simulink model "ElevatorPlant_Storage_A"  (R2015b)
(part 5 of 8)

            (junction 89650) -> (junction 89649)
            (junction 89651) -> (junction 89650)
          state Max_Min_assignment
            state Min_but
              en:
              BUTTON=MIN_BUT;
            state Max_but
              en:
              BUTTON=MAX_BUT;
            state First_but
              en:
              BUTTON=BUT_1;
            state Max_but1
              en:
              MAX_BUT=2;
            state Max_but2
              en:
              MAX_BUT=1;
            state Max_but3
              en:
              MAX_BUT=0;
            state Min_but1
              en:
              MIN_BUT=1;
            state Min_but2
              en:
              MIN_BUT=2;
            state Min_but3
              en:
              MIN_BUT=3;
            state MAX
              en:
              MAX_BUT=BUT_TEMP;
            state MIN
              en:
              MIN_BUT=BUT_TEMP;
            state Updating_button_0
              en:
              BUTTON=MAX_BUT;
            state Updating_button_1
              en:
              BUTTON=MIN_BUT;
            (junction 89689) -> OpCl_doors.OpCl_2.Opening2.Button_detection.Max_Min_assignment.Min_but [order 1] : [(MAX_BUT-FLOOR)>(FLOOR-MIN_BUT)]
            OpCl_doors.OpCl_2.Opening2.Button_detection.Max_Min_assignment.Min_but -> (junction 89690)
            (junction 89691) -> (junction 89689) [order 1] : [not(FLAG_STOP) && MOTION==2 && FLAG==3]
            (default) -> (junction 89691)
            (junction 89689) -> (junction 89692) [order 2]
            (junction 89690) -> (junction 89693)
            (junction 89691) -> (junction 89694) [order 2]
            (junction 89692) -> OpCl_doors.OpCl_2.Opening2.Button_detection.Max_Min_assignment.Max_but [order 1] : [(MAX_BUT-FLOOR)<(FLOOR-MIN_BUT)]
            OpCl_doors.OpCl_2.Opening2.Button_detection.Max_Min_assignment.Max_but -> (junction 89693)
            (junction 89692) -> OpCl_doors.OpCl_2.Opening2.Button_detection.Max_Min_assignment.First_but [order 2]
            (junction 89693) -> (junction 89696)
            OpCl_doors.OpCl_2.Opening2.Button_detection.Max_Min_assignment.First_but -> (junction 89695)
            (junction 89695) -> (junction 89694)
            (junction 89696) -> (junction 89695)
            (junction 89694) -> (junction 89697)
            (junction 89698) -> (junction 89699) [order 1] : [MOTION==0]
                | {MOTION=1;
                | UPDATE=true;}
            (junction 89699) -> OpCl_doors.OpCl_2.Opening2.Button_detection.Max_Min_assignment.Max_but1 [order 1] : [BUTTON_UP(2)]
            OpCl_doors.OpCl_2.Opening2.Button_detection.Max_Min_assignment.Max_but1 -> (junction 89700)
            (junction 89697) -> (junction 89698) [order 1] : [BUTTON==FLOOR && EXTEND]
                | {EXTEND=false;}
            (junction 89697) -> (junction 89711) [order 2]
            (junction 89698) -> (junction 89703) [order 2]
            (junction 89699) -> (junction 89701) [order 2]
            (junction 89700) -> (junction 89702)
            (junction 89701) -> OpCl_doors.OpCl_2.Opening2.Button_detection.Max_Min_assignment.Max_but2 [order 1] : [BUTTON_UP(1)]
            OpCl_doors.OpCl_2.Opening2.Button_detection.Max_Min_assignment.Max_but2 -> (junction 89702)
            (junction 89701) -> OpCl_doors.OpCl_2.Opening2.Button_detection.Max_Min_assignment.Max_but3 [order 2]
            (junction 89702) -> (junction 89705)
            OpCl_doors.OpCl_2.Opening2.Button_detection.Max_Min_assignment.Max_but3 -> (junction 89704)
            (junction 89704) -> (junction 89703)
            (junction 89705) -> (junction 89704)
            (junction 89703) -> (junction 89706)
            (junction 89706) -> (junction 89707) [order 1] : [MOTION==1]
                | {MOTION=0;
                | UPDATE=true;}
            (junction 89707) -> OpCl_doors.OpCl_2.Opening2.Button_detection.Max_Min_assignment.Min_but1 [order 1] : [BUTTON_DOWN(1)]
            OpCl_doors.OpCl_2.Opening2.Button_detection.Max_Min_assignment.Min_but1 -> (junction 89708)
            (junction 89706) -> (junction 89712) [order 2]
            (junction 89707) -> (junction 89709) [order 2]
            (junction 89708) -> (junction 89710)
            (junction 89709) -> OpCl_doors.OpCl_2.Opening2.Button_detection.Max_Min_assignment.Min_but2 [order 1] : [BUTTON_DOWN(2)]
            OpCl_doors.OpCl_2.Opening2.Button_detection.Max_Min_assignment.Min_but2 -> (junction 89710)
            (junction 89709) -> OpCl_doors.OpCl_2.Opening2.Button_detection.Max_Min_assignment.Min_but3 [order 2]
            (junction 89710) -> (junction 89714)
            OpCl_doors.OpCl_2.Opening2.Button_detection.Max_Min_assignment.Min_but3 -> (junction 89713)
            (junction 89712) -> (junction 89711)
            (junction 89713) -> (junction 89712)
            (junction 89714) -> (junction 89713)
            (junction 89711) -> (junction 89716)
            OpCl_doors.OpCl_2.Opening2.Button_detection.Max_Min_assignment.MAX -> (junction 89715)
            (junction 89716) -> (junction 89717) [order 1] : [PUSHED]
            (junction 89717) -> (junction 89718) [order 1] : [not(BUT_TEMP==FLOOR) || not(MOTION==2)]
            (junction 89718) -> OpCl_doors.OpCl_2.Opening2.Button_detection.Max_Min_assignment.MAX [order 1] : [MAX_BUT<BUT_TEMP && not(UPDATE)]
            (junction 89715) -> (junction 89720)
            (junction 89716) -> (junction 89730) [order 2]
            (junction 89717) -> (junction 89723) [order 2]
            (junction 89718) -> (junction 89719) [order 2]
            (junction 89720) -> (junction 89719)
            (junction 89719) -> (junction 89721)
            (junction 89721) -> OpCl_doors.OpCl_2.Opening2.Button_detection.Max_Min_assignment.MIN [order 1] : [MIN_BUT>BUT_TEMP && not(UPDATE)]
            OpCl_doors.OpCl_2.Opening2.Button_detection.Max_Min_assignment.MIN -> (junction 89722)
            (junction 89721) -> (junction 89724) [order 2]
            (junction 89722) -> (junction 89725)
            (junction 89724) -> (junction 89723)
            (junction 89725) -> (junction 89724)
            (junction 89723) -> (junction 89726)
            (junction 89726) -> OpCl_doors.OpCl_2.Opening2.Button_detection.Max_Min_assignment.Updating_button_0 [order 1] : [MOTION==0]
            OpCl_doors.OpCl_2.Opening2.Button_detection.Max_Min_assignment.Updating_button_0 -> (junction 89727)
            (junction 89726) -> (junction 89728) [order 2]
            (junction 89727) -> (junction 89729)
            (junction 89728) -> OpCl_doors.OpCl_2.Opening2.Button_detection.Max_Min_assignment.Updating_button_1 [order 1] : [MOTION==1]
            OpCl_doors.OpCl_2.Opening2.Button_detection.Max_Min_assignment.Updating_button_1 -> (junction 89729)
            (junction 89728) -> (junction 89731) [order 2]
            (junction 89729) -> (junction 89732)
            (junction 89731) -> (junction 89730)
            (junction 89732) -> (junction 89731)
          state GoTo_PositionControl
            en:
            BUTTON=BUT_TEMP;
            FLAG=2;
          state Emergency
            en:
            FLAG_EMG=true;
            FLAG=4;
          state Timer_EME
            state Set_tmr
              en:
              Q_EME=true;
            state Counting
              en:
              ET_EME= ET_EME + 1;
              Q_EME=false;
            state Set
              en:
              IN_EME=true;
              PT_EME=3;
            (junction 89822) -> OpCl_doors.OpCl_2.Opening2.Button_detection.Timer_EME.Set_tmr [order 1] : [ET_EME==PT_EME]
            OpCl_doors.OpCl_2.Opening2.Button_detection.Timer_EME.Set_tmr -> (junction 89823)
            OpCl_doors.OpCl_2.Opening2.Button_detection.Timer_EME.Counting -> (junction 89822)
            (junction 89822) -> (junction 89823) [order 2]
            (default) -> OpCl_doors.OpCl_2.Opening2.Button_detection.Timer_EME.Set
            OpCl_doors.OpCl_2.Opening2.Button_detection.Timer_EME.Set -> (junction 89824)
            (junction 89824) -> OpCl_doors.OpCl_2.Opening2.Button_detection.Timer_EME.Counting [order 1] : [ET_EME<PT_EME]
            (junction 89824) -> (junction 89823) [order 2]
          state Not_Emergency
            en:
            IN_EME=false;
            ET_EME=0;
          state SwitchingOFF_LEDs
            en:
            LPD3=false;
            LPD2=false;
            LPS2=false;
            LPD1=false;
            LPS1=false;
            LPS0=false;
          (default) -> (junction 89423)
          (junction 89423) -> (junction 89424) [order 1] : [FLAG==1 && not(PUSHED)]
              | {BUTTON=FLOOR;
              | BUT_TEMP=BUTTON;
              | BUT_1=FLOOR;}
          (junction 89424) -> OpCl_doors.OpCl_2.Opening2.Button_detection.Timer_LL [order 1] : [not(FLAG_STOP)]
          OpCl_doors.OpCl_2.Opening2.Button_detection.Timer_LL -> OpCl_doors.OpCl_2.Opening2.Button_detection.Save_energy
          OpCl_doors.OpCl_2.Opening2.Button_detection.Save_energy -> (junction 89425)
          (junction 89423) -> (junction 89426) [order 2]
          (junction 89424) -> (junction 89427) [order 2]
          (junction 89425) -> (junction 89428)
          (junction 89427) -> (junction 89426)
          (junction 89428) -> (junction 89427)
          (junction 89426) -> OpCl_doors.OpCl_2.Opening2.Button_detection.BUTTON_CAR
          OpCl_doors.OpCl_2.Opening2.Button_detection.BUTTON_UP -> OpCl_doors.OpCl_2.Opening2.Button_detection.BUTTON_DOWN
          OpCl_doors.OpCl_2.Opening2.Button_detection.BUTTON_DOWN -> OpCl_doors.OpCl_2.Opening2.Button_detection.Max_Min_assignment
          OpCl_doors.OpCl_2.Opening2.Button_detection.Max_Min_assignment -> (junction 89429)
          OpCl_doors.OpCl_2.Opening2.Button_detection.BUTTON_CAR -> OpCl_doors.OpCl_2.Opening2.Button_detection.BUTTON_UP
          (junction 89429) -> (junction 89431)
          (junction 89431) -> (junction 89430)
          (junction 89430) -> (junction 89432)
          (junction 89432) -> (junction 89433) [order 1] : [FLAG==1]
          (junction 89433) -> OpCl_doors.OpCl_2.Opening2.Button_detection.GoTo_PositionControl [order 1] : [PUSHED]
          OpCl_doors.OpCl_2.Opening2.Button_detection.GoTo_PositionControl -> (junction 89434)
          (junction 89432) -> (junction 89444) [order 2]
          (junction 89433) -> (junction 89435) [order 2]
          (junction 89434) -> (junction 89436)
          (junction 89436) -> (junction 89435)
          (junction 89435) -> (junction 89438)
          OpCl_doors.OpCl_2.Opening2.Button_detection.Emergency -> (junction 89437)
          (junction 89438) -> OpCl_doors.OpCl_2.Opening2.Button_detection.Timer_EME [order 1] : [STOP]
              | {IN_LL=false; ET_LL=0;FLAG=1;}
          OpCl_doors.OpCl_2.Opening2.Button_detection.Timer_EME -> (junction 89439)
          (junction 89439) -> OpCl_doors.OpCl_2.Opening2.Button_detection.Emergency [order 1] : [Q_EME]
          (junction 89437) -> (junction 89441)
          (junction 89438) -> OpCl_doors.OpCl_2.Opening2.Button_detection.Not_Emergency [order 2]
          (junction 89439) -> (junction 89440) [order 2]
          (junction 89441) -> (junction 89440)
          (junction 89440) -> (junction 89443)
          OpCl_doors.OpCl_2.Opening2.Button_detection.Not_Emergency -> (junction 89443)
          OpCl_doors.OpCl_2.Opening2.Button_detection.SwitchingOFF_LEDs -> (junction 89442)
          (junction 89443) -> OpCl_doors.OpCl_2.Opening2.Button_detection.SwitchingOFF_LEDs [order 1] : [FLAG_STOP && FLAG==2]
          (junction 89442) -> (junction 89446)
          (junction 89443) -> (junction 89445) [order 2]
          (junction 89445) -> (junction 89444)
          (junction 89446) -> (junction 89445)
        state Button_detection1
          state Save_energy
            en:
            LL=not(Q_LL);
          state Timer_LL
            state Set_tmr
              en:
              Q_LL=true;
            state Counting
              en:
              ET_LL= ET_LL + 1;
              Q_LL=false;
            state Set
              en:
              IN_LL=true;
              PT_LL=10;
            (junction 89907) -> OpCl_doors.OpCl_2.Opening2.Button_detection1.Timer_LL.Set_tmr [order 1] : [ET_LL==PT_LL]
            OpCl_doors.OpCl_2.Opening2.Button_detection1.Timer_LL.Set_tmr -> (junction 89908)
            OpCl_doors.OpCl_2.Opening2.Button_detection1.Timer_LL.Counting -> (junction 89907)
            (junction 89907) -> (junction 89908) [order 2]
            (default) -> OpCl_doors.OpCl_2.Opening2.Button_detection1.Timer_LL.Set
            OpCl_doors.OpCl_2.Opening2.Button_detection1.Timer_LL.Set -> (junction 89909)
            (junction 89909) -> OpCl_doors.OpCl_2.Opening2.Button_detection1.Timer_LL.Counting [order 1] : [ET_LL<PT_LL]
            (junction 89909) -> (junction 89908) [order 2]
          state BUTTON_DOWN
            state Button_DOWN_1
              en:
              BUTTON_DOWN(2)=true;
              BUT_TEMP=1;
              LPD1=true;
              PUSHED=true;
              UPDATE=false;
              IN_LL=false; ET_LL=0;
            state First_but_1
              en:
              BUT_1=BUT_TEMP;
              FIRST_BUT=false;
            state Button_DOWN_2
              en:
              BUTTON_DOWN(3)=true;
              BUT_TEMP=2;
              LPD2=true;
              PUSHED=true;
              UPDATE=false;
              IN_LL=false; ET_LL=0;
            state First_but_2
              en:
              BUT_1=BUT_TEMP;
              FIRST_BUT=false;
            state Button_DOWN_3
              en:
              BUTTON_DOWN(4)=true;
              BUT_TEMP=3;
              LPD3=true;
              PUSHED=true;
              UPDATE=false;
              IN_LL=false; ET_LL=0;
            state First_but_3
              en:
              BUT_1=BUT_TEMP;
              FIRST_BUT=false;
            (default) -> (junction 89922)
            (junction 89922) -> OpCl_doors.OpCl_2.Opening2.Button_detection1.BUTTON_DOWN.Button_DOWN_1 [order 1] : [PD1]
            OpCl_doors.OpCl_2.Opening2.Button_detection1.BUTTON_DOWN.Button_DOWN_1 -> (junction 89923)
            (junction 89923) -> OpCl_doors.OpCl_2.Opening2.Button_detection1.BUTTON_DOWN.First_but_1 [order 1] : [FIRST_BUT && not(RPC1)]
            OpCl_doors.OpCl_2.Opening2.Button_detection1.BUTTON_DOWN.First_but_1 -> (junction 89924)
            (junction 89922) -> (junction 89925) [order 2]
            (junction 89923) -> (junction 89926) [order 2]
            (junction 89924) -> (junction 89927)
            (junction 89926) -> (junction 89925)
            (junction 89927) -> (junction 89926)
            (junction 89925) -> (junction 89928)
            (junction 89928) -> OpCl_doors.OpCl_2.Opening2.Button_detection1.BUTTON_DOWN.Button_DOWN_2 [order 1] : [PD2]
            OpCl_doors.OpCl_2.Opening2.Button_detection1.BUTTON_DOWN.Button_DOWN_2 -> (junction 89929)
            (junction 89929) -> OpCl_doors.OpCl_2.Opening2.Button_detection1.BUTTON_DOWN.First_but_2 [order 1] : [FIRST_BUT && not(RPC2)]
            OpCl_doors.OpCl_2.Opening2.Button_detection1.BUTTON_DOWN.First_but_2 -> (junction 89930)
            (junction 89928) -> (junction 89931) [order 2]
            (junction 89929) -> (junction 89932) [order 2]
            (junction 89930) -> (junction 89933)
            (junction 89932) -> (junction 89931)
            (junction 89933) -> (junction 89932)
            (junction 89931) -> (junction 89934)
            (junction 89934) -> OpCl_doors.OpCl_2.Opening2.Button_detection1.BUTTON_DOWN.Button_DOWN_3 [order 1] : [PD3]
            OpCl_doors.OpCl_2.Opening2.Button_detection1.BUTTON_DOWN.Button_DOWN_3 -> (junction 89935)
            (junction 89935) -> OpCl_doors.OpCl_2.Opening2.Button_detection1.BUTTON_DOWN.First_but_3 [order 1] : [FIRST_BUT && not(RPC3)]
            OpCl_doors.OpCl_2.Opening2.Button_detection1.BUTTON_DOWN.First_but_3 -> (junction 89936)
            (junction 89934) -> (junction 89937) [order 2]
            (junction 89935) -> (junction 89938) [order 2]
            (junction 89936) -> (junction 89939)
            (junction 89938) -> (junction 89937)
            (junction 89939) -> (junction 89938)
          state BUTTON_CAR
            state Button_CAR_0
              en:
              BUTTON_CAR(1)=true;
              BUT_TEMP=0;
              LPC0=true;
              PUSHED=true;
              UPDATE=false;
              IN_LL=false; ET_LL=0;
            state First_but_0
              en:
              BUT_1=BUT_TEMP;
              FIRST_BUT=false;
            state Button_CAR_1
              en:
              BUTTON_CAR(2)=true;
              BUT_TEMP=1;
              LPC1=true;
              PUSHED=true;
              UPDATE=false;
              IN_LL=false; ET_LL=0;
            state First_but_1
              en:
              BUT_1=BUT_TEMP;
              FIRST_BUT=false;
            state Button_CAR_2
              en:
              BUTTON_CAR(3)=true;
              BUT_TEMP=2;
              LPC2=true;
              PUSHED=true;
              UPDATE=false;
              IN_LL=false; ET_LL=0;
            state First_but_2
              en:
              BUT_1=BUT_TEMP;
              FIRST_BUT=false;
            state Button_CAR_3
              en:
              BUTTON_CAR(4)=true;
              BUT_TEMP=3;
              LPC3=true;
              PUSHED=true;
              UPDATE=false;
              IN_LL=false; ET_LL=0;
            state First_but_3
              en:
              BUT_1=BUT_TEMP;
              FIRST_BUT=false;
            (default) -> (junction 89977)
            (junction 89977) -> OpCl_doors.OpCl_2.Opening2.Button_detection1.BUTTON_CAR.Button_CAR_0 [order 1] : [P0]
            OpCl_doors.OpCl_2.Opening2.Button_detection1.BUTTON_CAR.Button_CAR_0 -> (junction 89978)
            (junction 89978) -> OpCl_doors.OpCl_2.Opening2.Button_detection1.BUTTON_CAR.First_but_0 [order 1] : [FIRST_BUT && not(RPC0)]
            OpCl_doors.OpCl_2.Opening2.Button_detection1.BUTTON_CAR.First_but_0 -> (junction 89979)
            (junction 89977) -> (junction 89980) [order 2]
            (junction 89978) -> (junction 89981) [order 2]
            (junction 89979) -> (junction 89982)
            (junction 89981) -> (junction 89980)
            (junction 89982) -> (junction 89981)
            (junction 89980) -> (junction 89985)
            OpCl_doors.OpCl_2.Opening2.Button_detection1.BUTTON_CAR.Button_CAR_1 -> (junction 89983)
            (junction 89983) -> OpCl_doors.OpCl_2.Opening2.Button_detection1.BUTTON_CAR.First_but_1 [order 1] : [FIRST_BUT && not(RPC1)]
            OpCl_doors.OpCl_2.Opening2.Button_detection1.BUTTON_CAR.First_but_1 -> (junction 89984)
            (junction 89983) -> (junction 89987) [order 2]
            (junction 89984) -> (junction 89988)
            (junction 89985) -> OpCl_doors.OpCl_2.Opening2.Button_detection1.BUTTON_CAR.Button_CAR_1 [order 1] : [P1]
            (junction 89985) -> (junction 89986) [order 2]
            (junction 89987) -> (junction 89986)
            (junction 89988) -> (junction 89987)
            (junction 89986) -> (junction 89989)
            (junction 89989) -> OpCl_doors.OpCl_2.Opening2.Button_detection1.BUTTON_CAR.Button_CAR_2 [order 1] : [P2]
            OpCl_doors.OpCl_2.Opening2.Button_detection1.BUTTON_CAR.Button_CAR_2 -> (junction 89990)
            (junction 89990) -> OpCl_doors.OpCl_2.Opening2.Button_detection1.BUTTON_CAR.First_but_2 [order 1] : [FIRST_BUT && not(RPC2)]
            OpCl_doors.OpCl_2.Opening2.Button_detection1.BUTTON_CAR.First_but_2 -> (junction 89991)
            (junction 89989) -> (junction 89992) [order 2]
            (junction 89990) -> (junction 89993) [order 2]
            (junction 89991) -> (junction 89994)
            (junction 89993) -> (junction 89992)
            (junction 89994) -> (junction 89993)
            (junction 89992) -> (junction 89995)
            (junction 89995) -> OpCl_doors.OpCl_2.Opening2.Button_detection1.BUTTON_CAR.Button_CAR_3 [order 1] : [P3]
            OpCl_doors.OpCl_2.Opening2.Button_detection1.BUTTON_CAR.Button_CAR_3 -> (junction 89996)
            (junction 89996) -> OpCl_doors.OpCl_2.Opening2.Button_detection1.BUTTON_CAR.First_but_3 [order 1] : [FIRST_BUT && not(RPC3)]
            OpCl_doors.OpCl_2.Opening2.Button_detection1.BUTTON_CAR.First_but_3 -> (junction 89997)
            (junction 89995) -> (junction 89998) [order 2]
            (junction 89996) -> (junction 89999) [order 2]
            (junction 89997) -> (junction 90000)
            (junction 89999) -> (junction 89998)
            (junction 90000) -> (junction 89999)
          state BUTTON_UP
            state Button_UP_0
              en:
              BUTTON_UP(1)=true;
              BUT_TEMP=0;
              LPS0=true;
              PUSHED=true;
              UPDATE=false;
              IN_LL=false; ET_LL=0;
            state First_but_0
              en:
              BUT_1=BUT_TEMP;
              FIRST_BUT=false;
            state Button_UP_1
              en:
              BUTTON_UP(2)=true;
              BUT_TEMP=1;
              LPS1=true;
              PUSHED=true;
              UPDATE=false;
              IN_LL=false; ET_LL=0;
            state First_but_1
              en:
              BUT_1=BUT_TEMP;
              FIRST_BUT=false;
            state Button_UP_2
              en:
              BUTTON_UP(3)=true;
              BUT_TEMP=2;
              LPS2=true;
              PUSHED=true;
              UPDATE=false;
              IN_LL=false; ET_LL=0;
            state First_but_2
              en:
              BUT_1=BUT_TEMP;
              FIRST_BUT=false;
            (junction 90050) -> OpCl_doors.OpCl_2.Opening2.Button_detection1.BUTTON_UP.Button_UP_0 [order 1] : [PS0]
            OpCl_doors.OpCl_2.Opening2.Button_detection1.BUTTON_UP.Button_UP_0 -> (junction 90051)
            (junction 90051) -> OpCl_doors.OpCl_2.Opening2.Button_detection1.BUTTON_UP.First_but_0 [order 1] : [FIRST_BUT && not(RPC0)]
            OpCl_doors.OpCl_2.Opening2.Button_detection1.BUTTON_UP.First_but_0 -> (junction 90052)
            (default) -> (junction 90050)
            (junction 90050) -> (junction 90055) [order 2]
            (junction 90051) -> (junction 90053) [order 2]
            (junction 90052) -> (junction 90054)
            (junction 90054) -> (junction 90053)
            (junction 90053) -> (junction 90055)
            (junction 90055) -> (junction 90056)
            (junction 90056) -> OpCl_doors.OpCl_2.Opening2.Button_detection1.BUTTON_UP.Button_UP_1 [order 1] : [PS1]
            OpCl_doors.OpCl_2.Opening2.Button_detection1.BUTTON_UP.Button_UP_1 -> (junction 90057)
            (junction 90057) -> OpCl_doors.OpCl_2.Opening2.Button_detection1.BUTTON_UP.First_but_1 [order 1] : [FIRST_BUT && not(RPC1)]
            OpCl_doors.OpCl_2.Opening2.Button_detection1.BUTTON_UP.First_but_1 -> (junction 90058)
            (junction 90056) -> (junction 90059) [order 2]
            (junction 90057) -> (junction 90060) [order 2]
            (junction 90058) -> (junction 90061)
            (junction 90060) -> (junction 90059)
            (junction 90061) -> (junction 90060)
            (junction 90059) -> (junction 90063)
            OpCl_doors.OpCl_2.Opening2.Button_detection1.BUTTON_UP.First_but_2 -> (junction 90062)
            (junction 90062) -> (junction 90067)
            (junction 90063) -> OpCl_doors.OpCl_2.Opening2.Button_detection1.BUTTON_UP.Button_UP_2 [order 1] : [PS2]
            OpCl_doors.OpCl_2.Opening2.Button_detection1.BUTTON_UP.Button_UP_2 -> (junction 90064)
            (junction 90064) -> OpCl_doors.OpCl_2.Opening2.Button_detection1.BUTTON_UP.First_but_2 [order 1] : [FIRST_BUT && not(RPC2)]
            (junction 90063) -> (junction 90065) [order 2]
            (junction 90064) -> (junction 90066) [order 2]
            (junction 90066) -> (junction 90065)
            (junction 90067) -> (junction 90066)
          state Max_Min_assignment
            state Min_but
              en:
              BUTTON=MIN_BUT;
            state Max_but
              en:
              BUTTON=MAX_BUT;
            state First_but
              en:
              BUTTON=BUT_1;
            state Max_but1
              en:
              MAX_BUT=2;
            state Max_but2
              en:
              MAX_BUT=1;
            state Max_but3
              en:
              MAX_BUT=0;
            state Min_but1
              en:
              MIN_BUT=1;
            state Min_but2
              en:
              MIN_BUT=2;
            state Min_but3
              en:
              MIN_BUT=3;
            state MAX
              en:
              MAX_BUT=BUT_TEMP;
            state MIN
              en:
              MIN_BUT=BUT_TEMP;
            state Updating_button_0
              en:
              BUTTON=MAX_BUT;
            state Updating_button_1
              en:
              BUTTON=MIN_BUT;
            (junction 90105) -> OpCl_doors.OpCl_2.Opening2.Button_detection1.Max_Min_assignment.Min_but [order 1] : [(MAX_BUT-FLOOR)>(FLOOR-MIN_BUT)]
            OpCl_doors.OpCl_2.Opening2.Button_detection1.Max_Min_assignment.Min_but -> (junction 90106)
            (junction 90107) -> (junction 90105) [order 1] : [not(FLAG_STOP) && MOTION==2 && FLAG==3]
            (default) -> (junction 90107)
            (junction 90105) -> (junction 90108) [order 2]
            (junction 90106) -> (junction 90109)
            (junction 90107) -> (junction 90110) [order 2]
            (junction 90108) -> OpCl_doors.OpCl_2.Opening2.Button_detection1.Max_Min_assignment.Max_but [order 1] : [(MAX_BUT-FLOOR)<(FLOOR-MIN_BUT)]
            OpCl_doors.OpCl_2.Opening2.Button_detection1.Max_Min_assignment.Max_but -> (junction 90109)
            (junction 90108) -> OpCl_doors.OpCl_2.Opening2.Button_detection1.Max_Min_assignment.First_but [order 2]
            (junction 90109) -> (junction 90112)
            OpCl_doors.OpCl_2.Opening2.Button_detection1.Max_Min_assignment.First_but -> (junction 90111)
            (junction 90111) -> (junction 90110)
            (junction 90112) -> (junction 90111)
            (junction 90110) -> (junction 90113)
            (junction 90114) -> (junction 90115) [order 1] : [MOTION==0]
                | {MOTION=1;
                | UPDATE=true;}
            (junction 90115) -> OpCl_doors.OpCl_2.Opening2.Button_detection1.Max_Min_assignment.Max_but1 [order 1] : [BUTTON_UP(2)]
            OpCl_doors.OpCl_2.Opening2.Button_detection1.Max_Min_assignment.Max_but1 -> (junction 90116)
            (junction 90113) -> (junction 90114) [order 1] : [BUTTON==FLOOR && EXTEND]
                | {EXTEND=false;}
            (junction 90113) -> (junction 90127) [order 2]
            (junction 90114) -> (junction 90119) [order 2]
            (junction 90115) -> (junction 90117) [order 2]
            (junction 90116) -> (junction 90118)
            (junction 90117) -> OpCl_doors.OpCl_2.Opening2.Button_detection1.Max_Min_assignment.Max_but2 [order 1] : [BUTTON_UP(1)]
            OpCl_doors.OpCl_2.Opening2.Button_detection1.Max_Min_assignment.Max_but2 -> (junction 90118)
            (junction 90117) -> OpCl_doors.OpCl_2.Opening2.Button_detection1.Max_Min_assignment.Max_but3 [order 2]
            (junction 90118) -> (junction 90121)
            OpCl_doors.OpCl_2.Opening2.Button_detection1.Max_Min_assignment.Max_but3 -> (junction 90120)
            (junction 90120) -> (junction 90119)
            (junction 90121) -> (junction 90120)
            (junction 90119) -> (junction 90122)
            (junction 90122) -> (junction 90123) [order 1] : [MOTION==1]
                | {MOTION=0;
                | UPDATE=true;}
            (junction 90123) -> OpCl_doors.OpCl_2.Opening2.Button_detection1.Max_Min_assignment.Min_but1 [order 1] : [BUTTON_DOWN(1)]
            OpCl_doors.OpCl_2.Opening2.Button_detection1.Max_Min_assignment.Min_but1 -> (junction 90124)
            (junction 90122) -> (junction 90128) [order 2]
            (junction 90123) -> (junction 90125) [order 2]
            (junction 90124) -> (junction 90126)
            (junction 90125) -> OpCl_doors.OpCl_2.Opening2.Button_detection1.Max_Min_assignment.Min_but2 [order 1] : [BUTTON_DOWN(2)]
            OpCl_doors.OpCl_2.Opening2.Button_detection1.Max_Min_assignment.Min_but2 -> (junction 90126)
            (junction 90125) -> OpCl_doors.OpCl_2.Opening2.Button_detection1.Max_Min_assignment.Min_but3 [order 2]
            (junction 90126) -> (junction 90130)
            OpCl_doors.OpCl_2.Opening2.Button_detection1.Max_Min_assignment.Min_but3 -> (junction 90129)
            (junction 90128) -> (junction 90127)
            (junction 90129) -> (junction 90128)
            (junction 90130) -> (junction 90129)
            (junction 90127) -> (junction 90132)
            OpCl_doors.OpCl_2.Opening2.Button_detection1.Max_Min_assignment.MAX -> (junction 90131)
            (junction 90132) -> (junction 90133) [order 1] : [PUSHED]
            (junction 90133) -> (junction 90134) [order 1] : [not(BUT_TEMP==FLOOR) || not(MOTION==2)]
            (junction 90134) -> OpCl_doors.OpCl_2.Opening2.Button_detection1.Max_Min_assignment.MAX [order 1] : [MAX_BUT<BUT_TEMP && not(UPDATE)]
            (junction 90131) -> (junction 90136)
            (junction 90132) -> (junction 90146) [order 2]
            (junction 90133) -> (junction 90139) [order 2]
            (junction 90134) -> (junction 90135) [order 2]
            (junction 90136) -> (junction 90135)
            (junction 90135) -> (junction 90137)
            (junction 90137) -> OpCl_doors.OpCl_2.Opening2.Button_detection1.Max_Min_assignment.MIN [order 1] : [MIN_BUT>BUT_TEMP && not(UPDATE)]
            OpCl_doors.OpCl_2.Opening2.Button_detection1.Max_Min_assignment.MIN -> (junction 90138)
            (junction 90137) -> (junction 90140) [order 2]
            (junction 90138) -> (junction 90141)
            (junction 90140) -> (junction 90139)
            (junction 90141) -> (junction 90140)
            (junction 90139) -> (junction 90142)
            (junction 90142) -> OpCl_doors.OpCl_2.Opening2.Button_detection1.Max_Min_assignment.Updating_button_0 [order 1] : [MOTION==0]
            OpCl_doors.OpCl_2.Opening2.Button_detection1.Max_Min_assignment.Updating_button_0 -> (junction 90143)
            (junction 90142) -> (junction 90144) [order 2]
            (junction 90143) -> (junction 90145)
            (junction 90144) -> OpCl_doors.OpCl_2.Opening2.Button_detection1.Max_Min_assignment.Updating_button_1 [order 1] : [MOTION==1]
            OpCl_doors.OpCl_2.Opening2.Button_detection1.Max_Min_assignment.Updating_button_1 -> (junction 90145)
            (junction 90144) -> (junction 90147) [order 2]
            (junction 90145) -> (junction 90148)
            (junction 90147) -> (junction 90146)
            (junction 90148) -> (junction 90147)
          state GoTo_PositionControl
            en:
            BUTTON=BUT_TEMP;
            FLAG=2;
          state Emergency
            en:
            FLAG_EMG=true;
            FLAG=4;
          state Timer_EME
            state Set_tmr
              en:
              Q_EME=true;
            state Counting
              en:
              ET_EME= ET_EME + 1;
              Q_EME=false;
            state Set
              en:
              IN_EME=true;
              PT_EME=3;
            (junction 90238) -> OpCl_doors.OpCl_2.Opening2.Button_detection1.Timer_EME.Set_tmr [order 1] : [ET_EME==PT_EME]
            OpCl_doors.OpCl_2.Opening2.Button_detection1.Timer_EME.Set_tmr -> (junction 90239)
            OpCl_doors.OpCl_2.Opening2.Button_detection1.Timer_EME.Counting -> (junction 90238)
            (junction 90238) -> (junction 90239) [order 2]
            (default) -> OpCl_doors.OpCl_2.Opening2.Button_detection1.Timer_EME.Set
            OpCl_doors.OpCl_2.Opening2.Button_detection1.Timer_EME.Set -> (junction 90240)
            (junction 90240) -> OpCl_doors.OpCl_2.Opening2.Button_detection1.Timer_EME.Counting [order 1] : [ET_EME<PT_EME]
            (junction 90240) -> (junction 90239) [order 2]
          state Not_Emergency
            en:
            IN_EME=false;
            ET_EME=0;
          state SwitchingOFF_LEDs
            en:
            LPD3=false;
            LPD2=false;
            LPS2=false;
            LPD1=false;
            LPS1=false;
            LPS0=false;
          (default) -> (junction 89839)
          (junction 89839) -> (junction 89840) [order 1] : [FLAG==1 && not(PUSHED)]
              | {BUTTON=FLOOR;
              | BUT_TEMP=BUTTON;
              | BUT_1=FLOOR;}
          (junction 89840) -> OpCl_doors.OpCl_2.Opening2.Button_detection1.Timer_LL [order 1] : [not(FLAG_STOP)]
          OpCl_doors.OpCl_2.Opening2.Button_detection1.Save_energy -> (junction 89841)
          OpCl_doors.OpCl_2.Opening2.Button_detection1.Timer_LL -> OpCl_doors.OpCl_2.Opening2.Button_detection1.Save_energy
          (junction 89840) -> (junction 89843) [order 2]
          (junction 89839) -> (junction 89842) [order 2]
          (junction 89841) -> (junction 89844)
          (junction 89843) -> (junction 89842)
          (junction 89844) -> (junction 89843)
          (junction 89842) -> OpCl_doors.OpCl_2.Opening2.Button_detection1.BUTTON_CAR
          OpCl_doors.OpCl_2.Opening2.Button_detection1.BUTTON_UP -> OpCl_doors.OpCl_2.Opening2.Button_detection1.BUTTON_DOWN
          OpCl_doors.OpCl_2.Opening2.Button_detection1.BUTTON_DOWN -> OpCl_doors.OpCl_2.Opening2.Button_detection1.Max_Min_assignment
          OpCl_doors.OpCl_2.Opening2.Button_detection1.Max_Min_assignment -> (junction 89845)
          OpCl_doors.OpCl_2.Opening2.Button_detection1.BUTTON_CAR -> OpCl_doors.OpCl_2.Opening2.Button_detection1.BUTTON_UP
          (junction 89845) -> (junction 89847)
          (junction 89847) -> (junction 89846)
          (junction 89846) -> (junction 89849)
          OpCl_doors.OpCl_2.Opening2.Button_detection1.GoTo_PositionControl -> (junction 89848)
          (junction 89849) -> (junction 89850) [order 1] : [FLAG==1]
          (junction 89850) -> OpCl_doors.OpCl_2.Opening2.Button_detection1.GoTo_PositionControl [order 1] : [PUSHED]
          (junction 89848) -> (junction 89852)
          (junction 89849) -> (junction 89860) [order 2]
          (junction 89850) -> (junction 89851) [order 2]
          (junction 89852) -> (junction 89851)
          (junction 89851) -> (junction 89854)
          OpCl_doors.OpCl_2.Opening2.Button_detection1.Emergency -> (junction 89853)
          (junction 89854) -> OpCl_doors.OpCl_2.Opening2.Button_detection1.Timer_EME [order 1] : [STOP]
              | {IN_LL=false; ET_LL=0;FLAG=1;}
          OpCl_doors.OpCl_2.Opening2.Button_detection1.Timer_EME -> (junction 89855)
          (junction 89855) -> OpCl_doors.OpCl_2.Opening2.Button_detection1.Emergency [order 1] : [Q_EME]
          (junction 89853) -> (junction 89857)
          (junction 89854) -> OpCl_doors.OpCl_2.Opening2.Button_detection1.Not_Emergency [order 2]
          (junction 89855) -> (junction 89856) [order 2]
          (junction 89857) -> (junction 89856)
          (junction 89856) -> (junction 89859)
          OpCl_doors.OpCl_2.Opening2.Button_detection1.Not_Emergency -> (junction 89859)
          OpCl_doors.OpCl_2.Opening2.Button_detection1.SwitchingOFF_LEDs -> (junction 89858)
          (junction 89859) -> OpCl_doors.OpCl_2.Opening2.Button_detection1.SwitchingOFF_LEDs [order 1] : [FLAG_STOP && FLAG==2]
          (junction 89858) -> (junction 89862)
          (junction 89859) -> (junction 89861) [order 2]
          (junction 89861) -> (junction 89860)
          (junction 89862) -> (junction 89861)
        state Opening1
          en:AP2=true;
        state Reset
          state Reset_0
            en:
            LPS0=false;
            BUTTON_CAR(1)=false;
            BUTTON_UP(1)=false;
          state Reset_1
            en:
            LPS1=false;
            LPD1=false;
            BUTTON_CAR(2)=false;
            BUTTON_UP(2)=false;
            BUTTON_DOWN(2)=false;
          state Reset_2
            en:
            LPS2=false;
            LPD2=false;
            BUTTON_CAR(3)=false;
            BUTTON_UP(3)=false;
            BUTTON_DOWN(3)=false;
          state Reset_3
            en:
            LPD3=false;
            BUTTON_CAR(4)=false;
            BUTTON_DOWN(4)=false;
          (default) -> (junction 90256)
          (junction 90256) -> OpCl_doors.OpCl_2.Opening2.Reset.Reset_0 [order 1] : [FLOOR==0]
          OpCl_doors.OpCl_2.Opening2.Reset.Reset_0 -> (junction 90257)
          (junction 90256) -> (junction 90258) [order 2]
          (junction 90257) -> (junction 90259)
          (junction 90258) -> OpCl_doors.OpCl_2.Opening2.Reset.Reset_1 [order 1] : [FLOOR==1]
          OpCl_doors.OpCl_2.Opening2.Reset.Reset_1 -> (junction 90259)
          (junction 90258) -> (junction 90260) [order 2]
          (junction 90259) -> (junction 90261)
          (junction 90260) -> OpCl_doors.OpCl_2.Opening2.Reset.Reset_2 [order 1] : [FLOOR==2]
          OpCl_doors.OpCl_2.Opening2.Reset.Reset_2 -> (junction 90261)
          (junction 90260) -> (junction 90262) [order 2]
          (junction 90261) -> (junction 90263)
          (junction 90262) -> OpCl_doors.OpCl_2.Opening2.Reset.Reset_3 [order 1] : [FLOOR==3]
          OpCl_doors.OpCl_2.Opening2.Reset.Reset_3 -> (junction 90263)
          (junction 90262) -> (junction 90264) [order 2]
          (junction 90263) -> (junction 90265)
          (junction 90265) -> (junction 90264)
        state Stop_Opening1
          en: AP2=false;
          FLAG_OD=true;
          IN_cl=false;
          ET_cl=0;
        (junction 89253) -> (junction 89254)
        (junction 89254) -> (junction 89255) [order 1] : [not(OBS) ]
        (junction 89257) -> OpCl_doors.OpCl_2.Opening2.Opening [order 1] : [not(PA2)]
        (junction 89255) -> (junction 89256) [order 2]
        (junction 89256) -> OpCl_doors.OpCl_2.Opening2.Timer_open
        OpCl_doors.OpCl_2.Opening2.Timer_open -> (junction 89257)
        (default) -> OpCl_doors.OpCl_2.Opening2.People_IN
        (junction 89254) -> (junction 89258) [order 2]
        (junction 89255) -> OpCl_doors.OpCl_2.Opening2.Button_detection [order 1] : [not(FLAG==4)]
        (junction 89260) -> (junction 89256)
        (junction 89262) -> (junction 89253)
        (junction 89257) -> OpCl_doors.OpCl_2.Opening2.Stop_Opening [order 2]
        OpCl_doors.OpCl_2.Opening2.People_IN -> OpCl_doors.OpCl_2.Opening2.People_OUT
        OpCl_doors.OpCl_2.Opening2.Opening -> (junction 89267)
        (junction 89258) -> (junction 89259) [order 2]
        (junction 89258) -> OpCl_doors.OpCl_2.Opening2.Button_detection1 [order 1] : [not(FLAG==4)]
        (junction 89259) -> (junction 89264)
        OpCl_doors.OpCl_2.Opening2.Button_detection -> (junction 89260)
        OpCl_doors.OpCl_2.Opening2.People_OUT -> (junction 89261)
        OpCl_doors.OpCl_2.Opening2.Button_detection1 -> (junction 89263)
        (junction 89264) -> (junction 89263)
        (junction 89261) -> (junction 89262) [order 2]
        (junction 89261) -> OpCl_doors.OpCl_2.Opening2.Reset [order 1] : [not(FLAG==4)]
        (junction 89263) -> (junction 89265)
        (junction 89271) -> (junction 89262)
        OpCl_doors.OpCl_2.Opening2.Stop_Opening -> (junction 89266)
        (junction 89265) -> OpCl_doors.OpCl_2.Opening2.Opening1 [order 1] : [not(PA2)]
        (junction 89265) -> OpCl_doors.OpCl_2.Opening2.Stop_Opening1 [order 2]
        (junction 89267) -> (junction 89266)
        (junction 89266) -> (junction 89269)
        OpCl_doors.OpCl_2.Opening2.Opening1 -> (junction 89268)
        OpCl_doors.OpCl_2.Opening2.Reset -> (junction 89270)
        OpCl_doors.OpCl_2.Opening2.Stop_Opening1 -> (junction 89268)
        (junction 89268) -> (junction 89269)
        (junction 89270) -> (junction 89271)
      (default) -> (junction 12875)
      (junction 12875) -> (junction 12874) [order 1] : [FLAG_OD]
      (junction 12874) -> OpCl_doors.OpCl_2.Closing2 [order 1] : [not(SWITCH) && not(STOP) && WEIGHT<=320 && not(PS2 || PD2 || P2)]
      OpCl_doors.OpCl_2.Closing2 -> (junction 30489)
      (junction 12875) -> OpCl_doors.OpCl_2.Opening2 [order 2]
      (junction 12874) -> OpCl_doors.OpCl_2.StopClosing [order 2]
      (junction 30489) -> (junction 30490)
      OpCl_doors.OpCl_2.StopClosing -> (junction 30487)
      (junction 30490) -> (junction 30487)
      (junction 30487) -> (junction 30488)
      OpCl_doors.OpCl_2.Opening2 -> (junction 30488)
    state OpCl_3
      state Closing3
        state Reset
          state Reset_0
            en:
            LPS0=false;
            BUTTON_CAR(1)=false;
            BUTTON_UP(1)=false;
          state Reset_1
            en:
            LPS1=false;
            LPD1=false;
            BUTTON_CAR(2)=false;
            BUTTON_UP(2)=false;
            BUTTON_DOWN(2)=false;
          state Reset_2
            en:
            LPS2=false;
            LPD2=false;
            BUTTON_CAR(3)=false;
            BUTTON_UP(3)=false;
            BUTTON_DOWN(3)=false;
          state Reset_3
            en:
            LPD3=false;
            BUTTON_CAR(4)=false;
            BUTTON_DOWN(4)=false;
          (default) -> (junction 70468)
          (junction 70468) -> OpCl_doors.OpCl_3.Closing3.Reset.Reset_0 [order 1] : [FLOOR==0]
          OpCl_doors.OpCl_3.Closing3.Reset.Reset_0 -> (junction 70469)
          (junction 70468) -> (junction 70470) [order 2]
          (junction 70469) -> (junction 70471)
          (junction 70470) -> OpCl_doors.OpCl_3.Closing3.Reset.Reset_1 [order 1] : [FLOOR==1]
          OpCl_doors.OpCl_3.Closing3.Reset.Reset_1 -> (junction 70471)
          (junction 70470) -> (junction 70472) [order 2]
          (junction 70471) -> (junction 70473)
          (junction 70472) -> OpCl_doors.OpCl_3.Closing3.Reset.Reset_2 [order 1] : [FLOOR==2]
          OpCl_doors.OpCl_3.Closing3.Reset.Reset_2 -> (junction 70473)
          (junction 70472) -> (junction 70474) [order 2]
          (junction 70473) -> (junction 70475)
          (junction 70474) -> OpCl_doors.OpCl_3.Closing3.Reset.Reset_3 [order 1] : [FLOOR==3]
          OpCl_doors.OpCl_3.Closing3.Reset.Reset_3 -> (junction 70475)
          (junction 70474) -> (junction 70476) [order 2]
          (junction 70475) -> (junction 70477)
          (junction 70477) -> (junction 70476)
        state Timer_close
          state Set_tmr
            en: Q_cl=true;
          state Set
            en:PT_cl=5;
            IN_cl=true;
          state Counting
            en:ET_cl = ET_cl + 1;
            Q_cl=false;
          (junction 70501) -> OpCl_doors.OpCl_3.Closing3.Timer_close.Set_tmr [order 1] : [ET_cl==PT_cl]
          OpCl_doors.OpCl_3.Closing3.Timer_close.Set_tmr -> (junction 70502)
          (default) -> OpCl_doors.OpCl_3.Closing3.Timer_close.Set
          OpCl_doors.OpCl_3.Closing3.Timer_close.Counting -> (junction 70501)
          (junction 70501) -> (junction 70502) [order 2]
          OpCl_doors.OpCl_3.Closing3.Timer_close.Set -> (junction 70503)
          (junction 70503) -> OpCl_doors.OpCl_3.Closing3.Timer_close.Counting [order 1] : [ET_cl<PT_cl]
          (junction 70503) -> (junction 70502) [order 2]
        state Closing
          en: CP2=Q_cl;
        state Button_detection
          state Save_energy
            en:
            LL=not(Q_LL);
          state Timer_LL
            state Set_tmr
              en:
              Q_LL=true;
            state Counting
              en:
              ET_LL= ET_LL + 1;
              Q_LL=false;
            state Set
              en:
              IN_LL=true;
              PT_LL=10;
            (junction 70585) -> OpCl_doors.OpCl_3.Closing3.Button_detection.Timer_LL.Set_tmr [order 1] : [ET_LL==PT_LL]
            OpCl_doors.OpCl_3.Closing3.Button_detection.Timer_LL.Set_tmr -> (junction 70586)
            OpCl_doors.OpCl_3.Closing3.Button_detection.Timer_LL.Counting -> (junction 70585)
            (junction 70585) -> (junction 70586) [order 2]
            (default) -> OpCl_doors.OpCl_3.Closing3.Button_detection.Timer_LL.Set
            OpCl_doors.OpCl_3.Closing3.Button_detection.Timer_LL.Set -> (junction 70587)
            (junction 70587) -> OpCl_doors.OpCl_3.Closing3.Button_detection.Timer_LL.Counting [order 1] : [ET_LL<PT_LL]
            (junction 70587) -> (junction 70586) [order 2]
          state BUTTON_DOWN
            state Button_DOWN_1
              en:
              BUTTON_DOWN(2)=true;
              BUT_TEMP=1;
              LPD1=true;
              PUSHED=true;
              UPDATE=false;
              IN_LL=false; ET_LL=0;
            state First_but_1
              en:
              BUT_1=BUT_TEMP;
              FIRST_BUT=false;
            state Button_DOWN_2
              en:
              BUTTON_DOWN(3)=true;
              BUT_TEMP=2;
              LPD2=true;
              PUSHED=true;
              UPDATE=false;
              IN_LL=false; ET_LL=0;
            state First_but_2
              en:
              BUT_1=BUT_TEMP;
              FIRST_BUT=false;
            state Button_DOWN_3
              en:
              BUTTON_DOWN(4)=true;
              BUT_TEMP=3;
              LPD3=true;
              PUSHED=true;
              UPDATE=false;
              IN_LL=false; ET_LL=0;
            state First_but_3
              en:
              BUT_1=BUT_TEMP;
              FIRST_BUT=false;
            (default) -> (junction 70600)
            (junction 70600) -> OpCl_doors.OpCl_3.Closing3.Button_detection.BUTTON_DOWN.Button_DOWN_1 [order 1] : [PD1]
            OpCl_doors.OpCl_3.Closing3.Button_detection.BUTTON_DOWN.Button_DOWN_1 -> (junction 70601)
            (junction 70601) -> OpCl_doors.OpCl_3.Closing3.Button_detection.BUTTON_DOWN.First_but_1 [order 1] : [FIRST_BUT && not(RPC1)]
            OpCl_doors.OpCl_3.Closing3.Button_detection.BUTTON_DOWN.First_but_1 -> (junction 70602)
            (junction 70600) -> (junction 70603) [order 2]
            (junction 70601) -> (junction 70604) [order 2]
            (junction 70602) -> (junction 70605)
            (junction 70604) -> (junction 70603)
            (junction 70605) -> (junction 70604)
            (junction 70603) -> (junction 70606)
            (junction 70606) -> OpCl_doors.OpCl_3.Closing3.Button_detection.BUTTON_DOWN.Button_DOWN_2 [order 1] : [PD2]
            OpCl_doors.OpCl_3.Closing3.Button_detection.BUTTON_DOWN.Button_DOWN_2 -> (junction 70607)
            (junction 70607) -> OpCl_doors.OpCl_3.Closing3.Button_detection.BUTTON_DOWN.First_but_2 [order 1] : [FIRST_BUT && not(RPC2)]
            OpCl_doors.OpCl_3.Closing3.Button_detection.BUTTON_DOWN.First_but_2 -> (junction 70608)
            (junction 70606) -> (junction 70609) [order 2]
            (junction 70607) -> (junction 70610) [order 2]
            (junction 70608) -> (junction 70611)
            (junction 70610) -> (junction 70609)
            (junction 70611) -> (junction 70610)
            (junction 70609) -> (junction 70612)
            (junction 70612) -> OpCl_doors.OpCl_3.Closing3.Button_detection.BUTTON_DOWN.Button_DOWN_3 [order 1] : [PD3]
            OpCl_doors.OpCl_3.Closing3.Button_detection.BUTTON_DOWN.Button_DOWN_3 -> (junction 70613)
            (junction 70613) -> OpCl_doors.OpCl_3.Closing3.Button_detection.BUTTON_DOWN.First_but_3 [order 1] : [FIRST_BUT && not(RPC3)]
            OpCl_doors.OpCl_3.Closing3.Button_detection.BUTTON_DOWN.First_but_3 -> (junction 70614)
            (junction 70612) -> (junction 70615) [order 2]
            (junction 70613) -> (junction 70616) [order 2]
            (junction 70614) -> (junction 70617)
            (junction 70616) -> (junction 70615)
            (junction 70617) -> (junction 70616)
          state BUTTON_CAR
            state Button_CAR_0
              en:
              BUTTON_CAR(1)=true;
              BUT_TEMP=0;
              LPC0=true;
              PUSHED=true;
              UPDATE=false;
              IN_LL=false; ET_LL=0;
            state First_but_0
              en:
              BUT_1=BUT_TEMP;
              FIRST_BUT=false;
            state Button_CAR_1
              en:
              BUTTON_CAR(2)=true;
              BUT_TEMP=1;
              LPC1=true;
              PUSHED=true;
              UPDATE=false;
              IN_LL=false; ET_LL=0;
            state First_but_1
              en:
              BUT_1=BUT_TEMP;
              FIRST_BUT=false;
            state Button_CAR_2
              en:
              BUTTON_CAR(3)=true;
              BUT_TEMP=2;
              LPC2=true;
              PUSHED=true;
              UPDATE=false;
              IN_LL=false; ET_LL=0;
            state First_but_2
              en:
              BUT_1=BUT_TEMP;
              FIRST_BUT=false;
            state Button_CAR_3
              en:
              BUTTON_CAR(4)=true;
              BUT_TEMP=3;
              LPC3=true;
              PUSHED=true;
              UPDATE=false;
              IN_LL=false; ET_LL=0;
            state First_but_3
              en:
              BUT_1=BUT_TEMP;
              FIRST_BUT=false;
            (default) -> (junction 70655)
            (junction 70655) -> OpCl_doors.OpCl_3.Closing3.Button_detection.BUTTON_CAR.Button_CAR_0 [order 1] : [P0]
            OpCl_doors.OpCl_3.Closing3.Button_detection.BUTTON_CAR.Button_CAR_0 -> (junction 70656)
            (junction 70656) -> OpCl_doors.OpCl_3.Closing3.Button_detection.BUTTON_CAR.First_but_0 [order 1] : [FIRST_BUT && not(RPC0)]
            OpCl_doors.OpCl_3.Closing3.Button_detection.BUTTON_CAR.First_but_0 -> (junction 70657)
            (junction 70655) -> (junction 70658) [order 2]
            (junction 70656) -> (junction 70659) [order 2]
            (junction 70657) -> (junction 70660)
            (junction 70659) -> (junction 70658)
            (junction 70660) -> (junction 70659)
            (junction 70658) -> (junction 70663)
            OpCl_doors.OpCl_3.Closing3.Button_detection.BUTTON_CAR.Button_CAR_1 -> (junction 70661)
            (junction 70661) -> OpCl_doors.OpCl_3.Closing3.Button_detection.BUTTON_CAR.First_but_1 [order 1] : [FIRST_BUT && not(RPC1)]
            OpCl_doors.OpCl_3.Closing3.Button_detection.BUTTON_CAR.First_but_1 -> (junction 70662)
            (junction 70661) -> (junction 70665) [order 2]
            (junction 70662) -> (junction 70666)
            (junction 70663) -> OpCl_doors.OpCl_3.Closing3.Button_detection.BUTTON_CAR.Button_CAR_1 [order 1] : [P1]
            (junction 70663) -> (junction 70664) [order 2]
            (junction 70665) -> (junction 70664)
            (junction 70666) -> (junction 70665)
            (junction 70664) -> (junction 70667)
            (junction 70667) -> OpCl_doors.OpCl_3.Closing3.Button_detection.BUTTON_CAR.Button_CAR_2 [order 1] : [P2]
            OpCl_doors.OpCl_3.Closing3.Button_detection.BUTTON_CAR.Button_CAR_2 -> (junction 70668)
            (junction 70668) -> OpCl_doors.OpCl_3.Closing3.Button_detection.BUTTON_CAR.First_but_2 [order 1] : [FIRST_BUT && not(RPC2)]
            OpCl_doors.OpCl_3.Closing3.Button_detection.BUTTON_CAR.First_but_2 -> (junction 70669)
            (junction 70667) -> (junction 70670) [order 2]
            (junction 70668) -> (junction 70671) [order 2]
            (junction 70669) -> (junction 70672)
            (junction 70671) -> (junction 70670)
            (junction 70672) -> (junction 70671)
            (junction 70670) -> (junction 70673)
            (junction 70673) -> OpCl_doors.OpCl_3.Closing3.Button_detection.BUTTON_CAR.Button_CAR_3 [order 1] : [P3]
            OpCl_doors.OpCl_3.Closing3.Button_detection.BUTTON_CAR.Button_CAR_3 -> (junction 70674)
            (junction 70674) -> OpCl_doors.OpCl_3.Closing3.Button_detection.BUTTON_CAR.First_but_3 [order 1] : [FIRST_BUT && not(RPC3)]
            OpCl_doors.OpCl_3.Closing3.Button_detection.BUTTON_CAR.First_but_3 -> (junction 70675)
            (junction 70673) -> (junction 70676) [order 2]
            (junction 70674) -> (junction 70677) [order 2]
            (junction 70675) -> (junction 70678)
            (junction 70677) -> (junction 70676)
            (junction 70678) -> (junction 70677)
          state BUTTON_UP
            state Button_UP_0
              en:
              BUTTON_UP(1)=true;
              BUT_TEMP=0;
              LPS0=true;
              PUSHED=true;
              UPDATE=false;
              IN_LL=false; ET_LL=0;
            state First_but_0
              en:
              BUT_1=BUT_TEMP;
              FIRST_BUT=false;
            state Button_UP_1
              en:
              BUTTON_UP(2)=true;
              BUT_TEMP=1;
              LPS1=true;
              PUSHED=true;
              UPDATE=false;
              IN_LL=false; ET_LL=0;
            state First_but_1
              en:
              BUT_1=BUT_TEMP;
              FIRST_BUT=false;
            state Button_UP_2
              en:
              BUTTON_UP(3)=true;
              BUT_TEMP=2;
              LPS2=true;
              PUSHED=true;
              UPDATE=false;
              IN_LL=false; ET_LL=0;
            state First_but_2
              en:
              BUT_1=BUT_TEMP;
              FIRST_BUT=false;
            (junction 70728) -> OpCl_doors.OpCl_3.Closing3.Button_detection.BUTTON_UP.Button_UP_0 [order 1] : [PS0]
            OpCl_doors.OpCl_3.Closing3.Button_detection.BUTTON_UP.Button_UP_0 -> (junction 70729)
            (junction 70729) -> OpCl_doors.OpCl_3.Closing3.Button_detection.BUTTON_UP.First_but_0 [order 1] : [FIRST_BUT && not(RPC0)]
            OpCl_doors.OpCl_3.Closing3.Button_detection.BUTTON_UP.First_but_0 -> (junction 70730)
            (default) -> (junction 70728)
            (junction 70728) -> (junction 70733) [order 2]
            (junction 70729) -> (junction 70731) [order 2]
            (junction 70730) -> (junction 70732)
            (junction 70732) -> (junction 70731)
            (junction 70731) -> (junction 70733)
            (junction 70733) -> (junction 70734)
            (junction 70734) -> OpCl_doors.OpCl_3.Closing3.Button_detection.BUTTON_UP.Button_UP_1 [order 1] : [PS1]
            OpCl_doors.OpCl_3.Closing3.Button_detection.BUTTON_UP.Button_UP_1 -> (junction 70735)
            (junction 70735) -> OpCl_doors.OpCl_3.Closing3.Button_detection.BUTTON_UP.First_but_1 [order 1] : [FIRST_BUT && not(RPC1)]
            OpCl_doors.OpCl_3.Closing3.Button_detection.BUTTON_UP.First_but_1 -> (junction 70736)
            (junction 70734) -> (junction 70737) [order 2]
            (junction 70735) -> (junction 70738) [order 2]
            (junction 70736) -> (junction 70739)
            (junction 70738) -> (junction 70737)
            (junction 70739) -> (junction 70738)
            (junction 70737) -> (junction 70741)
            OpCl_doors.OpCl_3.Closing3.Button_detection.BUTTON_UP.First_but_2 -> (junction 70740)
            (junction 70740) -> (junction 70745)
            (junction 70741) -> OpCl_doors.OpCl_3.Closing3.Button_detection.BUTTON_UP.Button_UP_2 [order 1] : [PS2]
            OpCl_doors.OpCl_3.Closing3.Button_detection.BUTTON_UP.Button_UP_2 -> (junction 70742)
            (junction 70742) -> OpCl_doors.OpCl_3.Closing3.Button_detection.BUTTON_UP.First_but_2 [order 1] : [FIRST_BUT && not(RPC2)]
            (junction 70741) -> (junction 70743) [order 2]
            (junction 70742) -> (junction 70744) [order 2]
            (junction 70744) -> (junction 70743)
            (junction 70745) -> (junction 70744)
          state Max_Min_assignment
            state Min_but
              en:
              BUTTON=MIN_BUT;
            state Max_but
              en:
              BUTTON=MAX_BUT;
            state First_but
              en:
              BUTTON=BUT_1;
            state Max_but1
              en:
              MAX_BUT=2;
            state Max_but2
              en:
              MAX_BUT=1;
            state Max_but3
              en:
              MAX_BUT=0;
            state Min_but1
              en:
              MIN_BUT=1;
            state Min_but2
              en:
              MIN_BUT=2;
            state Min_but3
              en:
              MIN_BUT=3;
            state MAX
              en:
              MAX_BUT=BUT_TEMP;
            state MIN
              en:
              MIN_BUT=BUT_TEMP;
            state Updating_button_0
              en:
              BUTTON=MAX_BUT;
            state Updating_button_1
              en:
              BUTTON=MIN_BUT;
            (junction 70783) -> OpCl_doors.OpCl_3.Closing3.Button_detection.Max_Min_assignment.Min_but [order 1] : [(MAX_BUT-FLOOR)>(FLOOR-MIN_BUT)]
            OpCl_doors.OpCl_3.Closing3.Button_detection.Max_Min_assignment.Min_but -> (junction 70784)
            (junction 70785) -> (junction 70783) [order 1] : [not(FLAG_STOP) && MOTION==2 && FLAG==3]
            (default) -> (junction 70785)
            (junction 70783) -> (junction 70786) [order 2]
            (junction 70784) -> (junction 70787)
            (junction 70785) -> (junction 70788) [order 2]
            (junction 70786) -> OpCl_doors.OpCl_3.Closing3.Button_detection.Max_Min_assignment.Max_but [order 1] : [(MAX_BUT-FLOOR)<(FLOOR-MIN_BUT)]
            OpCl_doors.OpCl_3.Closing3.Button_detection.Max_Min_assignment.Max_but -> (junction 70787)
            (junction 70786) -> OpCl_doors.OpCl_3.Closing3.Button_detection.Max_Min_assignment.First_but [order 2]
            (junction 70787) -> (junction 70790)
            OpCl_doors.OpCl_3.Closing3.Button_detection.Max_Min_assignment.First_but -> (junction 70789)
            (junction 70789) -> (junction 70788)
            (junction 70790) -> (junction 70789)
            (junction 70788) -> (junction 70791)
            (junction 70792) -> (junction 70793) [order 1] : [MOTION==0]
                | {MOTION=1;
                | UPDATE=true;}
            (junction 70793) -> OpCl_doors.OpCl_3.Closing3.Button_detection.Max_Min_assignment.Max_but1 [order 1] : [BUTTON_UP(2)]
            OpCl_doors.OpCl_3.Closing3.Button_detection.Max_Min_assignment.Max_but1 -> (junction 70794)
            (junction 70791) -> (junction 70792) [order 1] : [BUTTON==FLOOR && EXTEND]
                | {EXTEND=false;}
            (junction 70791) -> (junction 70805) [order 2]
            (junction 70792) -> (junction 70797) [order 2]
            (junction 70793) -> (junction 70795) [order 2]
            (junction 70794) -> (junction 70796)
            (junction 70795) -> OpCl_doors.OpCl_3.Closing3.Button_detection.Max_Min_assignment.Max_but2 [order 1] : [BUTTON_UP(1)]
            OpCl_doors.OpCl_3.Closing3.Button_detection.Max_Min_assignment.Max_but2 -> (junction 70796)
            (junction 70795) -> OpCl_doors.OpCl_3.Closing3.Button_detection.Max_Min_assignment.Max_but3 [order 2]
            (junction 70796) -> (junction 70799)
            OpCl_doors.OpCl_3.Closing3.Button_detection.Max_Min_assignment.Max_but3 -> (junction 70798)
            (junction 70798) -> (junction 70797)
            (junction 70799) -> (junction 70798)
            (junction 70797) -> (junction 70800)
            (junction 70800) -> (junction 70801) [order 1] : [MOTION==1]
                | {MOTION=0;
                | UPDATE=true;}
            (junction 70801) -> OpCl_doors.OpCl_3.Closing3.Button_detection.Max_Min_assignment.Min_but1 [order 1] : [BUTTON_DOWN(1)]
            OpCl_doors.OpCl_3.Closing3.Button_detection.Max_Min_assignment.Min_but1 -> (junction 70802)
            (junction 70800) -> (junction 70806) [order 2]
            (junction 70801) -> (junction 70803) [order 2]
            (junction 70802) -> (junction 70804)
            (junction 70803) -> OpCl_doors.OpCl_3.Closing3.Button_detection.Max_Min_assignment.Min_but2 [order 1] : [BUTTON_DOWN(2)]
            OpCl_doors.OpCl_3.Closing3.Button_detection.Max_Min_assignment.Min_but2 -> (junction 70804)
            (junction 70803) -> OpCl_doors.OpCl_3.Closing3.Button_detection.Max_Min_assignment.Min_but3 [order 2]
            (junction 70804) -> (junction 70808)
            OpCl_doors.OpCl_3.Closing3.Button_detection.Max_Min_assignment.Min_but3 -> (junction 70807)
            (junction 70806) -> (junction 70805)
            (junction 70807) -> (junction 70806)
            (junction 70808) -> (junction 70807)
            (junction 70805) -> (junction 70810)
            OpCl_doors.OpCl_3.Closing3.Button_detection.Max_Min_assignment.MAX -> (junction 70809)
            (junction 70810) -> (junction 70811) [order 1] : [PUSHED]
            (junction 70811) -> (junction 70812) [order 1] : [not(BUT_TEMP==FLOOR) || not(MOTION==2)]
            (junction 70812) -> OpCl_doors.OpCl_3.Closing3.Button_detection.Max_Min_assignment.MAX [order 1] : [MAX_BUT<BUT_TEMP && not(UPDATE)]
            (junction 70809) -> (junction 70814)
            (junction 70810) -> (junction 70824) [order 2]
            (junction 70811) -> (junction 70817) [order 2]
            (junction 70812) -> (junction 70813) [order 2]
            (junction 70814) -> (junction 70813)
            (junction 70813) -> (junction 70815)
            (junction 70815) -> OpCl_doors.OpCl_3.Closing3.Button_detection.Max_Min_assignment.MIN [order 1] : [MIN_BUT>BUT_TEMP && not(UPDATE)]
            OpCl_doors.OpCl_3.Closing3.Button_detection.Max_Min_assignment.MIN -> (junction 70816)
            (junction 70815) -> (junction 70818) [order 2]
            (junction 70816) -> (junction 70819)
            (junction 70818) -> (junction 70817)
            (junction 70819) -> (junction 70818)
            (junction 70817) -> (junction 70820)
            (junction 70820) -> OpCl_doors.OpCl_3.Closing3.Button_detection.Max_Min_assignment.Updating_button_0 [order 1] : [MOTION==0]
            OpCl_doors.OpCl_3.Closing3.Button_detection.Max_Min_assignment.Updating_button_0 -> (junction 70821)
            (junction 70820) -> (junction 70822) [order 2]
            (junction 70821) -> (junction 70823)
            (junction 70822) -> OpCl_doors.OpCl_3.Closing3.Button_detection.Max_Min_assignment.Updating_button_1 [order 1] : [MOTION==1]
            OpCl_doors.OpCl_3.Closing3.Button_detection.Max_Min_assignment.Updating_button_1 -> (junction 70823)
            (junction 70822) -> (junction 70825) [order 2]
            (junction 70823) -> (junction 70826)
            (junction 70825) -> (junction 70824)
            (junction 70826) -> (junction 70825)
          state GoTo_PositionControl
            en:
            BUTTON=BUT_TEMP;
            FLAG=2;
          state Emergency
            en:
            FLAG_EMG=true;
            FLAG=4;
          state Timer_EME
            state Set_tmr
              en:
              Q_EME=true;
            state Counting
              en:
              ET_EME= ET_EME + 1;
              Q_EME=false;
            state Set
              en:
              IN_EME=true;
              PT_EME=3;
            (junction 70916) -> OpCl_doors.OpCl_3.Closing3.Button_detection.Timer_EME.Set_tmr [order 1] : [ET_EME==PT_EME]
            OpCl_doors.OpCl_3.Closing3.Button_detection.Timer_EME.Set_tmr -> (junction 70917)
            OpCl_doors.OpCl_3.Closing3.Button_detection.Timer_EME.Counting -> (junction 70916)
            (junction 70916) -> (junction 70917) [order 2]
            (default) -> OpCl_doors.OpCl_3.Closing3.Button_detection.Timer_EME.Set
            OpCl_doors.OpCl_3.Closing3.Button_detection.Timer_EME.Set -> (junction 70918)
            (junction 70918) -> OpCl_doors.OpCl_3.Closing3.Button_detection.Timer_EME.Counting [order 1] : [ET_EME<PT_EME]
            (junction 70918) -> (junction 70917) [order 2]
          state Not_Emergency
            en:
            IN_EME=false;
            ET_EME=0;
          state SwitchingOFF_LEDs
            en:
            LPD3=false;
            LPD2=false;
            LPS2=false;
            LPD1=false;
            LPS1=false;
            LPS0=false;
          (default) -> (junction 70517)
          (junction 70517) -> (junction 70518) [order 1] : [FLAG==1 && not(PUSHED)]
              | {BUTTON=FLOOR;
              | BUT_TEMP=BUTTON;
              | BUT_1=FLOOR;}
          (junction 70518) -> OpCl_doors.OpCl_3.Closing3.Button_detection.Timer_LL [order 1] : [not(FLAG_STOP)]
          OpCl_doors.OpCl_3.Closing3.Button_detection.Save_energy -> (junction 70519)
          OpCl_doors.OpCl_3.Closing3.Button_detection.Timer_LL -> OpCl_doors.OpCl_3.Closing3.Button_detection.Save_energy
          (junction 70518) -> (junction 70521) [order 2]
          (junction 70517) -> (junction 70520) [order 2]
          (junction 70519) -> (junction 70522)
          (junction 70521) -> (junction 70520)
          (junction 70522) -> (junction 70521)
          (junction 70520) -> OpCl_doors.OpCl_3.Closing3.Button_detection.BUTTON_CAR
          OpCl_doors.OpCl_3.Closing3.Button_detection.BUTTON_UP -> OpCl_doors.OpCl_3.Closing3.Button_detection.BUTTON_DOWN
          OpCl_doors.OpCl_3.Closing3.Button_detection.BUTTON_DOWN -> OpCl_doors.OpCl_3.Closing3.Button_detection.Max_Min_assignment
          OpCl_doors.OpCl_3.Closing3.Button_detection.Max_Min_assignment -> (junction 70523)
          OpCl_doors.OpCl_3.Closing3.Button_detection.BUTTON_CAR -> OpCl_doors.OpCl_3.Closing3.Button_detection.BUTTON_UP
          (junction 70523) -> (junction 70525)
          (junction 70525) -> (junction 70524)
          (junction 70524) -> (junction 70527)
          OpCl_doors.OpCl_3.Closing3.Button_detection.GoTo_PositionControl -> (junction 70526)
          (junction 70527) -> (junction 70528) [order 1] : [FLAG==1]
          (junction 70528) -> OpCl_doors.OpCl_3.Closing3.Button_detection.GoTo_PositionControl [order 1] : [PUSHED]
          (junction 70526) -> (junction 70530)
          (junction 70527) -> (junction 70538) [order 2]
          (junction 70528) -> (junction 70529) [order 2]
          (junction 70530) -> (junction 70529)
          (junction 70529) -> (junction 70532)
          OpCl_doors.OpCl_3.Closing3.Button_detection.Emergency -> (junction 70531)
          (junction 70532) -> OpCl_doors.OpCl_3.Closing3.Button_detection.Timer_EME [order 1] : [STOP]
              | {IN_LL=false; ET_LL=0;FLAG=1;}
          OpCl_doors.OpCl_3.Closing3.Button_detection.Timer_EME -> (junction 70533)
          (junction 70533) -> OpCl_doors.OpCl_3.Closing3.Button_detection.Emergency [order 1] : [Q_EME]
          (junction 70531) -> (junction 70535)
          (junction 70532) -> OpCl_doors.OpCl_3.Closing3.Button_detection.Not_Emergency [order 2]
          (junction 70533) -> (junction 70534) [order 2]
          (junction 70535) -> (junction 70534)
          (junction 70534) -> (junction 70537)
          OpCl_doors.OpCl_3.Closing3.Button_detection.Not_Emergency -> (junction 70537)
          OpCl_doors.OpCl_3.Closing3.Button_detection.SwitchingOFF_LEDs -> (junction 70536)
          (junction 70537) -> OpCl_doors.OpCl_3.Closing3.Button_detection.SwitchingOFF_LEDs [order 1] : [FLAG_STOP && FLAG==2]
          (junction 70536) -> (junction 70540)
          (junction 70537) -> (junction 70539) [order 2]
          (junction 70539) -> (junction 70538)
          (junction 70540) -> (junction 70539)
        state Extending
          en:
          EXTEND=true;
        state Stop_Closing
          en:
          CP2=false;
          FLAG_OD=false;
          OBS=false;
          ET_cl=0;
          IN_cl=false;
        state GoTo_PositionControl
          en: FLAG=2;
        state GoTo_BUttonDetection
          en:
          MOTION=2;
          MAX_BUT=0;
          MIN_BUT=3;
          PUSHED=false;
          FIRST_BUT=true;
          FLAG=1;
          UPDATE=false;
        state Closing1
          en:CP2=true;
        state Stop_Closing1
          en:CP2=false;
        OpCl_doors.OpCl_3.Closing3.Reset -> OpCl_doors.OpCl_3.Closing3.Timer_close
        (default) -> (junction 70428)
        (junction 70428) -> OpCl_doors.OpCl_3.Closing3.Reset [order 1] : [not(FLAG==0) && not(FLAG==4)]
        OpCl_doors.OpCl_3.Closing3.Timer_close -> (junction 70429)
        (junction 70429) -> OpCl_doors.OpCl_3.Closing3.Closing [order 1] : [not(PC2)]
        OpCl_doors.OpCl_3.Closing3.Button_detection -> (junction 70430)
        OpCl_doors.OpCl_3.Closing3.Closing -> OpCl_doors.OpCl_3.Closing3.Button_detection
        (junction 70428) -> (junction 70438) [order 2]
        (junction 70429) -> (junction 70431) [order 2]
        (junction 70430) -> (junction 70436)
        (junction 70431) -> OpCl_doors.OpCl_3.Closing3.Extending [order 1] : [BUTTON==FLOOR]
        (junction 70431) -> (junction 70433) [order 2]
        OpCl_doors.OpCl_3.Closing3.Extending -> (junction 70432)
        (junction 70432) -> (junction 70433)
        (junction 70433) -> OpCl_doors.OpCl_3.Closing3.Stop_Closing
        OpCl_doors.OpCl_3.Closing3.Stop_Closing -> (junction 70434)
        (junction 70434) -> OpCl_doors.OpCl_3.Closing3.GoTo_PositionControl [order 2]
        (junction 70434) -> OpCl_doors.OpCl_3.Closing3.GoTo_BUttonDetection [order 1] : [not(BUTTON_CAR(1) || BUTTON_CAR(2) || BUTTON_CAR(3) || BUTTON_CAR(4) || BUTTON_UP(1) || BUTTON_UP(2) || BUTTON_UP(3) || BUTTON_DOWN(2) || BUTTON_DOWN(3) || BUTTON_DOWN(4))]
        OpCl_doors.OpCl_3.Closing3.GoTo_PositionControl -> (junction 70435)
        OpCl_doors.OpCl_3.Closing3.GoTo_BUttonDetection -> (junction 70435)
        (junction 70435) -> (junction 70436)
        (junction 70436) -> (junction 70437)
        (junction 70437) -> (junction 70439)
        (junction 70438) -> OpCl_doors.OpCl_3.Closing3.Closing1 [order 1] : [not(PC2)]
        OpCl_doors.OpCl_3.Closing3.Closing1 -> (junction 70439)
        (junction 70438) -> OpCl_doors.OpCl_3.Closing3.Stop_Closing1 [order 2]
        OpCl_doors.OpCl_3.Closing3.Stop_Closing1 -> (junction 70439)
      state StopClosing
        en: CP3=false;
        FLAG_OD=false;
      state Opening3
        state Opening
          en:AP3=Q_op;
        state People_IN
          state Check_People_IN
            en:
            COUNTER_IN=false;
          state People_KID_IN
            en:
            WEIGHT=WEIGHT+30;
            KIDS=KIDS+1;
          state People_WOMAN_IN
            en:
            WEIGHT=WEIGHT+55;
            WOMEN=WOMEN+1;
          state People_MAN_IN
            en:
            WEIGHT=WEIGHT+75;
            MEN=MEN+1;
          state People_FATGUY_IN
            en:
            WEIGHT=WEIGHT+100;
            FATGUYS=FATGUYS+1;
          state Re_Ready_IN
            en:
            COUNTER_IN=true;
          (default) -> (junction 90346)
          (junction 90346) -> OpCl_doors.OpCl_3.Opening3.People_IN.Check_People_IN [order 1] : [COUNTER_IN]
          OpCl_doors.OpCl_3.Opening3.People_IN.Check_People_IN -> (junction 90347)
          (junction 90347) -> OpCl_doors.OpCl_3.Opening3.People_IN.People_KID_IN [order 1] : [KID_IN]
          OpCl_doors.OpCl_3.Opening3.People_IN.People_KID_IN -> (junction 90348)
          (junction 90346) -> (junction 90355) [order 2]
          (junction 90347) -> (junction 90349) [order 2]
          (junction 90348) -> (junction 90350)
          (junction 90349) -> OpCl_doors.OpCl_3.Opening3.People_IN.People_WOMAN_IN [order 1] : [WOMAN_IN]
          OpCl_doors.OpCl_3.Opening3.People_IN.People_WOMAN_IN -> (junction 90350)
          (junction 90349) -> (junction 90351) [order 2]
          (junction 90350) -> (junction 90352)
          (junction 90351) -> OpCl_doors.OpCl_3.Opening3.People_IN.People_MAN_IN [order 1] : [MAN_IN]
          OpCl_doors.OpCl_3.Opening3.People_IN.People_MAN_IN -> (junction 90352)
          (junction 90351) -> (junction 90353) [order 2]
          (junction 90352) -> (junction 90354)
          (junction 90353) -> OpCl_doors.OpCl_3.Opening3.People_IN.People_FATGUY_IN [order 1] : [FATGUY_IN]
          OpCl_doors.OpCl_3.Opening3.People_IN.People_FATGUY_IN -> (junction 90354)
          (junction 90353) -> (junction 90356) [order 2]
          (junction 90354) -> (junction 90357)
          (junction 90356) -> (junction 90355)
          (junction 90357) -> (junction 90356)
          (junction 90355) -> (junction 90358)
          (junction 90358) -> OpCl_doors.OpCl_3.Opening3.People_IN.Re_Ready_IN [order 1] : [not(KID_IN|| WOMAN_IN || MAN_IN || FATGUY_IN)]
          (junction 90358) -> (junction 90359) [order 2]
          OpCl_doors.OpCl_3.Opening3.People_IN.Re_Ready_IN -> (junction 90360)
          (junction 90360) -> (junction 90359)
        state Timer_open
          state Set_tmr
            en: Q_op=true;
          state Set
            en:PT_op=2;
            IN_op=true;
          state Counting
            en:ET_op = ET_op + 1;
            Q_op=false;
          (junction 90395) -> OpCl_doors.OpCl_3.Opening3.Timer_open.Set_tmr [order 1] : [ET_op==PT_op]
          OpCl_doors.OpCl_3.Opening3.Timer_open.Set_tmr -> (junction 90396)
          (default) -> OpCl_doors.OpCl_3.Opening3.Timer_open.Set
          OpCl_doors.OpCl_3.Opening3.Timer_open.Counting -> (junction 90395)
          (junction 90395) -> (junction 90396) [order 2]
          OpCl_doors.OpCl_3.Opening3.Timer_open.Set -> (junction 90397)
          (junction 90397) -> OpCl_doors.OpCl_3.Opening3.Timer_open.Counting [order 1] : [ET_op<PT_op]
          (junction 90397) -> (junction 90396) [order 2]
        state Stop_Opening
          en:AP3=false;
          FLAG_OD=true;
          OBS=true;
          IN_op=false;
          ET_op=0;
        state People_OUT
          state Check_People_OUT
            en:
            COUNTER_OUT=false;
          state People_KID_OUT
            en:
            WEIGHT=WEIGHT-30;
            KIDS=KIDS-1;
          state People_WOMAN_OUT
            en:
            WEIGHT=WEIGHT-55;
            WOMEN=WOMEN-1;
          state People_MAN_OUT
            en:
            WEIGHT=WEIGHT-75;
            MEN=MEN-1;
          state People_FATGUY_OUT
            en:
            WEIGHT=WEIGHT-100;
            FATGUYS=FATGUYS-1;
          state Re_Ready_OUT
            en:
            COUNTER_OUT=true;
          (default) -> (junction 90411)
          (junction 90411) -> OpCl_doors.OpCl_3.Opening3.People_OUT.Check_People_OUT [order 1] : [COUNTER_OUT]
          OpCl_doors.OpCl_3.Opening3.People_OUT.Check_People_OUT -> (junction 90412)
          (junction 90412) -> OpCl_doors.OpCl_3.Opening3.People_OUT.People_KID_OUT [order 1] : [KID_OUT && KIDS>0 ]
          OpCl_doors.OpCl_3.Opening3.People_OUT.People_KID_OUT -> (junction 90413)
          (junction 90411) -> (junction 90420) [order 2]
          (junction 90412) -> (junction 90414) [order 2]
          (junction 90413) -> (junction 90415)
          (junction 90414) -> OpCl_doors.OpCl_3.Opening3.People_OUT.People_WOMAN_OUT [order 1] : [WOMAN_OUT && WOMEN>0]
          OpCl_doors.OpCl_3.Opening3.People_OUT.People_WOMAN_OUT -> (junction 90415)
          (junction 90415) -> (junction 90417)
          (junction 90414) -> (junction 90416) [order 2]
          (junction 90416) -> OpCl_doors.OpCl_3.Opening3.People_OUT.People_MAN_OUT [order 1] : [MAN_OUT && MEN>0]
          OpCl_doors.OpCl_3.Opening3.People_OUT.People_MAN_OUT -> (junction 90417)
          (junction 90416) -> (junction 90418) [order 2]
          (junction 90417) -> (junction 90419)
          (junction 90418) -> OpCl_doors.OpCl_3.Opening3.People_OUT.People_FATGUY_OUT [order 1] : [FATGUY_OUT && FATGUYS>0]
          OpCl_doors.OpCl_3.Opening3.People_OUT.People_FATGUY_OUT -> (junction 90419)
          (junction 90418) -> (junction 90421) [order 2]
          (junction 90419) -> (junction 90422)
          (junction 90421) -> (junction 90420)
          (junction 90422) -> (junction 90421)
          (junction 90420) -> (junction 90423)
          (junction 90423) -> OpCl_doors.OpCl_3.Opening3.People_OUT.Re_Ready_OUT [order 1] : [not(KID_OUT || WOMAN_OUT || MAN_OUT || FATGUY_OUT)]
          (junction 90423) -> (junction 90424) [order 2]
          OpCl_doors.OpCl_3.Opening3.People_OUT.Re_Ready_OUT -> (junction 90425)
          (junction 90425) -> (junction 90424)
        state Button_detection
          state Save_energy
            en:
            LL=not(Q_LL);
          state Timer_LL
            state Set_tmr
              en:
              Q_LL=true;
            state Counting
              en:
              ET_LL= ET_LL + 1;
              Q_LL=false;
            state Set
              en:
              IN_LL=true;
              PT_LL=10;
            (junction 90528) -> OpCl_doors.OpCl_3.Opening3.Button_detection.Timer_LL.Set_tmr [order 1] : [ET_LL==PT_LL]
            OpCl_doors.OpCl_3.Opening3.Button_detection.Timer_LL.Set_tmr -> (junction 90529)
            OpCl_doors.OpCl_3.Opening3.Button_detection.Timer_LL.Counting -> (junction 90528)
            (junction 90528) -> (junction 90529) [order 2]
            (default) -> OpCl_doors.OpCl_3.Opening3.Button_detection.Timer_LL.Set
            OpCl_doors.OpCl_3.Opening3.Button_detection.Timer_LL.Set -> (junction 90530)
            (junction 90530) -> OpCl_doors.OpCl_3.Opening3.Button_detection.Timer_LL.Counting [order 1] : [ET_LL<PT_LL]
            (junction 90530) -> (junction 90529) [order 2]
          state BUTTON_DOWN
            state Button_DOWN_1
              en:
              BUTTON_DOWN(2)=true;
              BUT_TEMP=1;
              LPD1=true;
              PUSHED=true;
              UPDATE=false;
              IN_LL=false; ET_LL=0;
            state First_but_1
              en:
              BUT_1=BUT_TEMP;
              FIRST_BUT=false;
            state Button_DOWN_2
              en:
              BUTTON_DOWN(3)=true;
              BUT_TEMP=2;
              LPD2=true;
              PUSHED=true;
              UPDATE=false;
              IN_LL=false; ET_LL=0;
            state First_but_2
              en:
              BUT_1=BUT_TEMP;
              FIRST_BUT=false;
            state Button_DOWN_3
              en:
              BUTTON_DOWN(4)=true;
              BUT_TEMP=3;
              LPD3=true;
              PUSHED=true;
              UPDATE=false;
              IN_LL=false; ET_LL=0;
            state First_but_3
              en:
              BUT_1=BUT_TEMP;
              FIRST_BUT=false;
            (default) -> (junction 90543)
            (junction 90543) -> OpCl_doors.OpCl_3.Opening3.Button_detection.BUTTON_DOWN.Button_DOWN_1 [order 1] : [PD1]
            OpCl_doors.OpCl_3.Opening3.Button_detection.BUTTON_DOWN.Button_DOWN_1 -> (junction 90544)
            (junction 90544) -> OpCl_doors.OpCl_3.Opening3.Button_detection.BUTTON_DOWN.First_but_1 [order 1] : [FIRST_BUT && not(RPC1)]
            OpCl_doors.OpCl_3.Opening3.Button_detection.BUTTON_DOWN.First_but_1 -> (junction 90545)
            (junction 90543) -> (junction 90546) [order 2]
            (junction 90544) -> (junction 90547) [order 2]
            (junction 90545) -> (junction 90548)
            (junction 90547) -> (junction 90546)
            (junction 90548) -> (junction 90547)
            (junction 90546) -> (junction 90549)
            (junction 90549) -> OpCl_doors.OpCl_3.Opening3.Button_detection.BUTTON_DOWN.Button_DOWN_2 [order 1] : [PD2]
            OpCl_doors.OpCl_3.Opening3.Button_detection.BUTTON_DOWN.Button_DOWN_2 -> (junction 90550)
            (junction 90550) -> OpCl_doors.OpCl_3.Opening3.Button_detection.BUTTON_DOWN.First_but_2 [order 1] : [FIRST_BUT && not(RPC2)]
            OpCl_doors.OpCl_3.Opening3.Button_detection.BUTTON_DOWN.First_but_2 -> (junction 90551)
            (junction 90549) -> (junction 90552) [order 2]
            (junction 90550) -> (junction 90553) [order 2]
            (junction 90551) -> (junction 90554)
            (junction 90553) -> (junction 90552)
            (junction 90554) -> (junction 90553)
            (junction 90552) -> (junction 90555)
            (junction 90555) -> OpCl_doors.OpCl_3.Opening3.Button_detection.BUTTON_DOWN.Button_DOWN_3 [order 1] : [PD3]
            OpCl_doors.OpCl_3.Opening3.Button_detection.BUTTON_DOWN.Button_DOWN_3 -> (junction 90556)
            (junction 90556) -> OpCl_doors.OpCl_3.Opening3.Button_detection.BUTTON_DOWN.First_but_3 [order 1] : [FIRST_BUT && not(RPC3)]
            OpCl_doors.OpCl_3.Opening3.Button_detection.BUTTON_DOWN.First_but_3 -> (junction 90557)
            (junction 90555) -> (junction 90558) [order 2]
            (junction 90556) -> (junction 90559) [order 2]
            (junction 90557) -> (junction 90560)
            (junction 90559) -> (junction 90558)
            (junction 90560) -> (junction 90559)
          state BUTTON_CAR
            state Button_CAR_0
              en:
              BUTTON_CAR(1)=true;
              BUT_TEMP=0;
              LPC0=true;
              PUSHED=true;
              UPDATE=false;
              IN_LL=false; ET_LL=0;
            state First_but_0
              en:
              BUT_1=BUT_TEMP;
              FIRST_BUT=false;
            state Button_CAR_1
              en:
              BUTTON_CAR(2)=true;
              BUT_TEMP=1;
              LPC1=true;
              PUSHED=true;
              UPDATE=false;
              IN_LL=false; ET_LL=0;
            state First_but_1
              en:
              BUT_1=BUT_TEMP;
              FIRST_BUT=false;
            state Button_CAR_2
              en:
              BUTTON_CAR(3)=true;
              BUT_TEMP=2;
              LPC2=true;
              PUSHED=true;
              UPDATE=false;
              IN_LL=false; ET_LL=0;
            state First_but_2
              en:
              BUT_1=BUT_TEMP;
              FIRST_BUT=false;
            state Button_CAR_3
              en:
              BUTTON_CAR(4)=true;
              BUT_TEMP=3;
              LPC3=true;
              PUSHED=true;
              UPDATE=false;
              IN_LL=false; ET_LL=0;
            state First_but_3
              en:
              BUT_1=BUT_TEMP;
              FIRST_BUT=false;
            (default) -> (junction 90598)
            (junction 90598) -> OpCl_doors.OpCl_3.Opening3.Button_detection.BUTTON_CAR.Button_CAR_0 [order 1] : [P0]
            OpCl_doors.OpCl_3.Opening3.Button_detection.BUTTON_CAR.Button_CAR_0 -> (junction 90599)
            (junction 90599) -> OpCl_doors.OpCl_3.Opening3.Button_detection.BUTTON_CAR.First_but_0 [order 1] : [FIRST_BUT && not(RPC0)]
            OpCl_doors.OpCl_3.Opening3.Button_detection.BUTTON_CAR.First_but_0 -> (junction 90600)
            (junction 90598) -> (junction 90601) [order 2]
            (junction 90599) -> (junction 90602) [order 2]
            (junction 90600) -> (junction 90603)
            (junction 90602) -> (junction 90601)
            (junction 90603) -> (junction 90602)
            (junction 90601) -> (junction 90606)
            OpCl_doors.OpCl_3.Opening3.Button_detection.BUTTON_CAR.Button_CAR_1 -> (junction 90604)
            (junction 90604) -> OpCl_doors.OpCl_3.Opening3.Button_detection.BUTTON_CAR.First_but_1 [order 1] : [FIRST_BUT && not(RPC1)]
            OpCl_doors.OpCl_3.Opening3.Button_detection.BUTTON_CAR.First_but_1 -> (junction 90605)
            (junction 90604) -> (junction 90608) [order 2]
            (junction 90605) -> (junction 90609)
            (junction 90606) -> OpCl_doors.OpCl_3.Opening3.Button_detection.BUTTON_CAR.Button_CAR_1 [order 1] : [P1]
            (junction 90606) -> (junction 90607) [order 2]
            (junction 90608) -> (junction 90607)
            (junction 90609) -> (junction 90608)
            (junction 90607) -> (junction 90610)
            (junction 90610) -> OpCl_doors.OpCl_3.Opening3.Button_detection.BUTTON_CAR.Button_CAR_2 [order 1] : [P2]
            OpCl_doors.OpCl_3.Opening3.Button_detection.BUTTON_CAR.Button_CAR_2 -> (junction 90611)
            (junction 90611) -> OpCl_doors.OpCl_3.Opening3.Button_detection.BUTTON_CAR.First_but_2 [order 1] : [FIRST_BUT && not(RPC2)]
            OpCl_doors.OpCl_3.Opening3.Button_detection.BUTTON_CAR.First_but_2 -> (junction 90612)
            (junction 90610) -> (junction 90613) [order 2]
            (junction 90611) -> (junction 90614) [order 2]
            (junction 90612) -> (junction 90615)
            (junction 90614) -> (junction 90613)
            (junction 90615) -> (junction 90614)
            (junction 90613) -> (junction 90616)
            (junction 90616) -> OpCl_doors.OpCl_3.Opening3.Button_detection.BUTTON_CAR.Button_CAR_3 [order 1] : [P3]
            OpCl_doors.OpCl_3.Opening3.Button_detection.BUTTON_CAR.Button_CAR_3 -> (junction 90617)
            (junction 90617) -> OpCl_doors.OpCl_3.Opening3.Button_detection.BUTTON_CAR.First_but_3 [order 1] : [FIRST_BUT && not(RPC3)]
            OpCl_doors.OpCl_3.Opening3.Button_detection.BUTTON_CAR.First_but_3 -> (junction 90618)
            (junction 90616) -> (junction 90619) [order 2]
            (junction 90617) -> (junction 90620) [order 2]
            (junction 90618) -> (junction 90621)
            (junction 90620) -> (junction 90619)
            (junction 90621) -> (junction 90620)
          state BUTTON_UP
            state Button_UP_0
              en:
              BUTTON_UP(1)=true;
              BUT_TEMP=0;
              LPS0=true;
              PUSHED=true;
              UPDATE=false;
              IN_LL=false; ET_LL=0;
            state First_but_0
              en:
              BUT_1=BUT_TEMP;
              FIRST_BUT=false;
            state Button_UP_1
              en:
              BUTTON_UP(2)=true;
              BUT_TEMP=1;
              LPS1=true;
              PUSHED=true;
              UPDATE=false;
              IN_LL=false; ET_LL=0;
            state First_but_1
              en:
              BUT_1=BUT_TEMP;
              FIRST_BUT=false;
            state Button_UP_2
              en:
              BUTTON_UP(3)=true;
              BUT_TEMP=2;
              LPS2=true;
              PUSHED=true;
              UPDATE=false;
              IN_LL=false; ET_LL=0;
            state First_but_2
              en:
              BUT_1=BUT_TEMP;
              FIRST_BUT=false;
            (junction 90671) -> OpCl_doors.OpCl_3.Opening3.Button_detection.BUTTON_UP.Button_UP_0 [order 1] : [PS0]
            OpCl_doors.OpCl_3.Opening3.Button_detection.BUTTON_UP.Button_UP_0 -> (junction 90672)
            (junction 90672) -> OpCl_doors.OpCl_3.Opening3.Button_detection.BUTTON_UP.First_but_0 [order 1] : [FIRST_BUT && not(RPC0)]
            OpCl_doors.OpCl_3.Opening3.Button_detection.BUTTON_UP.First_but_0 -> (junction 90673)
            (default) -> (junction 90671)
            (junction 90671) -> (junction 90676) [order 2]
            (junction 90672) -> (junction 90674) [order 2]
            (junction 90673) -> (junction 90675)
            (junction 90675) -> (junction 90674)
            (junction 90674) -> (junction 90676)
            (junction 90676) -> (junction 90677)
            (junction 90677) -> OpCl_doors.OpCl_3.Opening3.Button_detection.BUTTON_UP.Button_UP_1 [order 1] : [PS1]
            OpCl_doors.OpCl_3.Opening3.Button_detection.BUTTON_UP.Button_UP_1 -> (junction 90678)
            (junction 90678) -> OpCl_doors.OpCl_3.Opening3.Button_detection.BUTTON_UP.First_but_1 [order 1] : [FIRST_BUT && not(RPC1)]
            OpCl_doors.OpCl_3.Opening3.Button_detection.BUTTON_UP.First_but_1 -> (junction 90679)
            (junction 90677) -> (junction 90680) [order 2]
            (junction 90678) -> (junction 90681) [order 2]
            (junction 90679) -> (junction 90682)
            (junction 90681) -> (junction 90680)
            (junction 90682) -> (junction 90681)
            (junction 90680) -> (junction 90684)
            OpCl_doors.OpCl_3.Opening3.Button_detection.BUTTON_UP.First_but_2 -> (junction 90683)
            (junction 90683) -> (junction 90688)
            (junction 90684) -> OpCl_doors.OpCl_3.Opening3.Button_detection.BUTTON_UP.Button_UP_2 [order 1] : [PS2]
            OpCl_doors.OpCl_3.Opening3.Button_detection.BUTTON_UP.Button_UP_2 -> (junction 90685)
            (junction 90685) -> OpCl_doors.OpCl_3.Opening3.Button_detection.BUTTON_UP.First_but_2 [order 1] : [FIRST_BUT && not(RPC2)]
            (junction 90684) -> (junction 90686) [order 2]
            (junction 90685) -> (junction 90687) [order 2]
            (junction 90687) -> (junction 90686)
            (junction 90688) -> (junction 90687)
          state Max_Min_assignment
            state Min_but
              en:
              BUTTON=MIN_BUT;
            state Max_but
              en:
              BUTTON=MAX_BUT;
            state First_but
              en:
              BUTTON=BUT_1;
            state Max_but1
              en:
              MAX_BUT=2;
            state Max_but2
              en:
              MAX_BUT=1;
            state Max_but3
              en:
              MAX_BUT=0;
            state Min_but1
              en:
              MIN_BUT=1;
            state Min_but2
              en:
              MIN_BUT=2;
            state Min_but3
              en:
              MIN_BUT=3;
            state MAX
              en:
              MAX_BUT=BUT_TEMP;
            state MIN
              en:
              MIN_BUT=BUT_TEMP;
            state Updating_button_0
              en:
              BUTTON=MAX_BUT;
            state Updating_button_1
              en:
              BUTTON=MIN_BUT;
            (junction 90726) -> OpCl_doors.OpCl_3.Opening3.Button_detection.Max_Min_assignment.Min_but [order 1] : [(MAX_BUT-FLOOR)>(FLOOR-MIN_BUT)]
            OpCl_doors.OpCl_3.Opening3.Button_detection.Max_Min_assignment.Min_but -> (junction 90727)
            (junction 90728) -> (junction 90726) [order 1] : [not(FLAG_STOP) && MOTION==2 && FLAG==3]
            (default) -> (junction 90728)
            (junction 90726) -> (junction 90729) [order 2]
            (junction 90727) -> (junction 90730)
            (junction 90728) -> (junction 90731) [order 2]
            (junction 90729) -> OpCl_doors.OpCl_3.Opening3.Button_detection.Max_Min_assignment.Max_but [order 1] : [(MAX_BUT-FLOOR)<(FLOOR-MIN_BUT)]
            OpCl_doors.OpCl_3.Opening3.Button_detection.Max_Min_assignment.Max_but -> (junction 90730)
            (junction 90729) -> OpCl_doors.OpCl_3.Opening3.Button_detection.Max_Min_assignment.First_but [order 2]
            (junction 90730) -> (junction 90733)
            OpCl_doors.OpCl_3.Opening3.Button_detection.Max_Min_assignment.First_but -> (junction 90732)
            (junction 90732) -> (junction 90731)
            (junction 90733) -> (junction 90732)
            (junction 90731) -> (junction 90734)
            (junction 90735) -> (junction 90736) [order 1] : [MOTION==0]
                | {MOTION=1;
                | UPDATE=true;}
            (junction 90736) -> OpCl_doors.OpCl_3.Opening3.Button_detection.Max_Min_assignment.Max_but1 [order 1] : [BUTTON_UP(2)]
            OpCl_doors.OpCl_3.Opening3.Button_detection.Max_Min_assignment.Max_but1 -> (junction 90737)
            (junction 90734) -> (junction 90735) [order 1] : [BUTTON==FLOOR && EXTEND]
                | {EXTEND=false;}
            (junction 90734) -> (junction 90748) [order 2]
            (junction 90735) -> (junction 90740) [order 2]
            (junction 90736) -> (junction 90738) [order 2]
            (junction 90737) -> (junction 90739)
            (junction 90738) -> OpCl_doors.OpCl_3.Opening3.Button_detection.Max_Min_assignment.Max_but2 [order 1] : [BUTTON_UP(1)]
            OpCl_doors.OpCl_3.Opening3.Button_detection.Max_Min_assignment.Max_but2 -> (junction 90739)
            (junction 90738) -> OpCl_doors.OpCl_3.Opening3.Button_detection.Max_Min_assignment.Max_but3 [order 2]
            (junction 90739) -> (junction 90742)
            OpCl_doors.OpCl_3.Opening3.Button_detection.Max_Min_assignment.Max_but3 -> (junction 90741)
            (junction 90741) -> (junction 90740)
            (junction 90742) -> (junction 90741)
            (junction 90740) -> (junction 90743)
            (junction 90743) -> (junction 90744) [order 1] : [MOTION==1]
                | {MOTION=0;
                | UPDATE=true;}
            (junction 90744) -> OpCl_doors.OpCl_3.Opening3.Button_detection.Max_Min_assignment.Min_but1 [order 1] : [BUTTON_DOWN(1)]
            OpCl_doors.OpCl_3.Opening3.Button_detection.Max_Min_assignment.Min_but1 -> (junction 90745)
            (junction 90743) -> (junction 90749) [order 2]
            (junction 90744) -> (junction 90746) [order 2]
            (junction 90745) -> (junction 90747)
            (junction 90746) -> OpCl_doors.OpCl_3.Opening3.Button_detection.Max_Min_assignment.Min_but2 [order 1] : [BUTTON_DOWN(2)]
            OpCl_doors.OpCl_3.Opening3.Button_detection.Max_Min_assignment.Min_but2 -> (junction 90747)
            (junction 90746) -> OpCl_doors.OpCl_3.Opening3.Button_detection.Max_Min_assignment.Min_but3 [order 2]
            (junction 90747) -> (junction 90751)
            OpCl_doors.OpCl_3.Opening3.Button_detection.Max_Min_assignment.Min_but3 -> (junction 90750)
            (junction 90749) -> (junction 90748)
            (junction 90750) -> (junction 90749)
            (junction 90751) -> (junction 90750)
            (junction 90748) -> (junction 90753)
            OpCl_doors.OpCl_3.Opening3.Button_detection.Max_Min_assignment.MAX -> (junction 90752)
            (junction 90753) -> (junction 90754) [order 1] : [PUSHED]
            (junction 90754) -> (junction 90755) [order 1] : [not(BUT_TEMP==FLOOR) || not(MOTION==2)]
            (junction 90755) -> OpCl_doors.OpCl_3.Opening3.Button_detection.Max_Min_assignment.MAX [order 1] : [MAX_BUT<BUT_TEMP && not(UPDATE)]
            (junction 90752) -> (junction 90757)
            (junction 90753) -> (junction 90767) [order 2]
            (junction 90754) -> (junction 90760) [order 2]
            (junction 90755) -> (junction 90756) [order 2]
            (junction 90757) -> (junction 90756)
            (junction 90756) -> (junction 90758)
            (junction 90758) -> OpCl_doors.OpCl_3.Opening3.Button_detection.Max_Min_assignment.MIN [order 1] : [MIN_BUT>BUT_TEMP && not(UPDATE)]
            OpCl_doors.OpCl_3.Opening3.Button_detection.Max_Min_assignment.MIN -> (junction 90759)
            (junction 90758) -> (junction 90761) [order 2]
            (junction 90759) -> (junction 90762)
            (junction 90761) -> (junction 90760)
            (junction 90762) -> (junction 90761)
            (junction 90760) -> (junction 90763)
            (junction 90763) -> OpCl_doors.OpCl_3.Opening3.Button_detection.Max_Min_assignment.Updating_button_0 [order 1] : [MOTION==0]
            OpCl_doors.OpCl_3.Opening3.Button_detection.Max_Min_assignment.Updating_button_0 -> (junction 90764)
            (junction 90763) -> (junction 90765) [order 2]
            (junction 90764) -> (junction 90766)
            (junction 90765) -> OpCl_doors.OpCl_3.Opening3.Button_detection.Max_Min_assignment.Updating_button_1 [order 1] : [MOTION==1]
            OpCl_doors.OpCl_3.Opening3.Button_detection.Max_Min_assignment.Updating_button_1 -> (junction 90766)
            (junction 90765) -> (junction 90768) [order 2]
            (junction 90766) -> (junction 90769)
            (junction 90768) -> (junction 90767)
            (junction 90769) -> (junction 90768)
          state GoTo_PositionControl
            en:
            BUTTON=BUT_TEMP;
            FLAG=2;
          state Emergency
            en:
            FLAG_EMG=true;
            FLAG=4;
          state Timer_EME
            state Set_tmr
              en:
              Q_EME=true;
            state Counting
              en:
              ET_EME= ET_EME + 1;
              Q_EME=false;
            state Set
              en:
              IN_EME=true;
              PT_EME=3;
            (junction 90859) -> OpCl_doors.OpCl_3.Opening3.Button_detection.Timer_EME.Set_tmr [order 1] : [ET_EME==PT_EME]
            OpCl_doors.OpCl_3.Opening3.Button_detection.Timer_EME.Set_tmr -> (junction 90860)
            OpCl_doors.OpCl_3.Opening3.Button_detection.Timer_EME.Counting -> (junction 90859)
            (junction 90859) -> (junction 90860) [order 2]
            (default) -> OpCl_doors.OpCl_3.Opening3.Button_detection.Timer_EME.Set
            OpCl_doors.OpCl_3.Opening3.Button_detection.Timer_EME.Set -> (junction 90861)
            (junction 90861) -> OpCl_doors.OpCl_3.Opening3.Button_detection.Timer_EME.Counting [order 1] : [ET_EME<PT_EME]
            (junction 90861) -> (junction 90860) [order 2]
          state Not_Emergency
            en:
            IN_EME=false;
            ET_EME=0;
          state SwitchingOFF_LEDs
            en:
            LPD3=false;
            LPD2=false;
            LPS2=false;
            LPD1=false;
            LPS1=false;
            LPS0=false;
          (default) -> (junction 90460)
          (junction 90460) -> (junction 90461) [order 1] : [FLAG==1 && not(PUSHED)]
              | {BUTTON=FLOOR;
              | BUT_TEMP=BUTTON;
              | BUT_1=FLOOR;}
          (junction 90461) -> OpCl_doors.OpCl_3.Opening3.Button_detection.Timer_LL [order 1] : [not(FLAG_STOP)]
          OpCl_doors.OpCl_3.Opening3.Button_detection.Timer_LL -> OpCl_doors.OpCl_3.Opening3.Button_detection.Save_energy
          OpCl_doors.OpCl_3.Opening3.Button_detection.Save_energy -> (junction 90462)
          (junction 90460) -> (junction 90463) [order 2]
          (junction 90461) -> (junction 90464) [order 2]
          (junction 90462) -> (junction 90465)
          (junction 90464) -> (junction 90463)
          (junction 90465) -> (junction 90464)
          (junction 90463) -> OpCl_doors.OpCl_3.Opening3.Button_detection.BUTTON_CAR
          OpCl_doors.OpCl_3.Opening3.Button_detection.BUTTON_UP -> OpCl_doors.OpCl_3.Opening3.Button_detection.BUTTON_DOWN
          OpCl_doors.OpCl_3.Opening3.Button_detection.BUTTON_DOWN -> OpCl_doors.OpCl_3.Opening3.Button_detection.Max_Min_assignment
          OpCl_doors.OpCl_3.Opening3.Button_detection.Max_Min_assignment -> (junction 90466)
          OpCl_doors.OpCl_3.Opening3.Button_detection.BUTTON_CAR -> OpCl_doors.OpCl_3.Opening3.Button_detection.BUTTON_UP
          (junction 90466) -> (junction 90468)
          (junction 90468) -> (junction 90467)
          (junction 90467) -> (junction 90469)
          (junction 90469) -> (junction 90470) [order 1] : [FLAG==1]
          (junction 90470) -> OpCl_doors.OpCl_3.Opening3.Button_detection.GoTo_PositionControl [order 1] : [PUSHED]
          OpCl_doors.OpCl_3.Opening3.Button_detection.GoTo_PositionControl -> (junction 90471)
          (junction 90469) -> (junction 90481) [order 2]
          (junction 90470) -> (junction 90472) [order 2]
          (junction 90471) -> (junction 90473)
          (junction 90473) -> (junction 90472)
          (junction 90472) -> (junction 90475)
          OpCl_doors.OpCl_3.Opening3.Button_detection.Emergency -> (junction 90474)
          (junction 90475) -> OpCl_doors.OpCl_3.Opening3.Button_detection.Timer_EME [order 1] : [STOP]
              | {IN_LL=false; ET_LL=0;FLAG=1;}
          OpCl_doors.OpCl_3.Opening3.Button_detection.Timer_EME -> (junction 90476)
          (junction 90476) -> OpCl_doors.OpCl_3.Opening3.Button_detection.Emergency [order 1] : [Q_EME]
          (junction 90474) -> (junction 90478)
          (junction 90475) -> OpCl_doors.OpCl_3.Opening3.Button_detection.Not_Emergency [order 2]
          (junction 90476) -> (junction 90477) [order 2]
          (junction 90478) -> (junction 90477)
          (junction 90477) -> (junction 90480)
          OpCl_doors.OpCl_3.Opening3.Button_detection.Not_Emergency -> (junction 90480)
          OpCl_doors.OpCl_3.Opening3.Button_detection.SwitchingOFF_LEDs -> (junction 90479)
          (junction 90480) -> OpCl_doors.OpCl_3.Opening3.Button_detection.SwitchingOFF_LEDs [order 1] : [FLAG_STOP && FLAG==2]
          (junction 90479) -> (junction 90483)
          (junction 90480) -> (junction 90482) [order 2]
          (junction 90482) -> (junction 90481)
          (junction 90483) -> (junction 90482)
        state Button_detection1
          state Save_energy
            en:
            LL=not(Q_LL);
          state Timer_LL
            state Set_tmr
              en:
              Q_LL=true;
            state Counting
              en:
              ET_LL= ET_LL + 1;
              Q_LL=false;
            state Set
              en:
              IN_LL=true;
              PT_LL=10;
            (junction 90944) -> OpCl_doors.OpCl_3.Opening3.Button_detection1.Timer_LL.Set_tmr [order 1] : [ET_LL==PT_LL]
            OpCl_doors.OpCl_3.Opening3.Button_detection1.Timer_LL.Set_tmr -> (junction 90945)
            OpCl_doors.OpCl_3.Opening3.Button_detection1.Timer_LL.Counting -> (junction 90944)
            (junction 90944) -> (junction 90945) [order 2]
            (default) -> OpCl_doors.OpCl_3.Opening3.Button_detection1.Timer_LL.Set
            OpCl_doors.OpCl_3.Opening3.Button_detection1.Timer_LL.Set -> (junction 90946)
            (junction 90946) -> OpCl_doors.OpCl_3.Opening3.Button_detection1.Timer_LL.Counting [order 1] : [ET_LL<PT_LL]
            (junction 90946) -> (junction 90945) [order 2]
          state BUTTON_DOWN
            state Button_DOWN_1
              en:
              BUTTON_DOWN(2)=true;
              BUT_TEMP=1;
              LPD1=true;
              PUSHED=true;
              UPDATE=false;
              IN_LL=false; ET_LL=0;
            state First_but_1
              en:
              BUT_1=BUT_TEMP;
              FIRST_BUT=false;
            state Button_DOWN_2
              en:
              BUTTON_DOWN(3)=true;
              BUT_TEMP=2;
              LPD2=true;
              PUSHED=true;
              UPDATE=false;
              IN_LL=false; ET_LL=0;
            state First_but_2
              en:
              BUT_1=BUT_TEMP;
              FIRST_BUT=false;
            state Button_DOWN_3
              en:
              BUTTON_DOWN(4)=true;
              BUT_TEMP=3;
              LPD3=true;
              PUSHED=true;
              UPDATE=false;
              IN_LL=false; ET_LL=0;
            state First_but_3
              en:
              BUT_1=BUT_TEMP;
              FIRST_BUT=false;
            (default) -> (junction 90959)
            (junction 90959) -> OpCl_doors.OpCl_3.Opening3.Button_detection1.BUTTON_DOWN.Button_DOWN_1 [order 1] : [PD1]
            OpCl_doors.OpCl_3.Opening3.Button_detection1.BUTTON_DOWN.Button_DOWN_1 -> (junction 90960)
            (junction 90960) -> OpCl_doors.OpCl_3.Opening3.Button_detection1.BUTTON_DOWN.First_but_1 [order 1] : [FIRST_BUT && not(RPC1)]
            OpCl_doors.OpCl_3.Opening3.Button_detection1.BUTTON_DOWN.First_but_1 -> (junction 90961)
            (junction 90959) -> (junction 90962) [order 2]
            (junction 90960) -> (junction 90963) [order 2]
            (junction 90961) -> (junction 90964)
            (junction 90963) -> (junction 90962)
            (junction 90964) -> (junction 90963)
            (junction 90962) -> (junction 90965)
            (junction 90965) -> OpCl_doors.OpCl_3.Opening3.Button_detection1.BUTTON_DOWN.Button_DOWN_2 [order 1] : [PD2]
            OpCl_doors.OpCl_3.Opening3.Button_detection1.BUTTON_DOWN.Button_DOWN_2 -> (junction 90966)
            (junction 90966) -> OpCl_doors.OpCl_3.Opening3.Button_detection1.BUTTON_DOWN.First_but_2 [order 1] : [FIRST_BUT && not(RPC2)]
            OpCl_doors.OpCl_3.Opening3.Button_detection1.BUTTON_DOWN.First_but_2 -> (junction 90967)
            (junction 90965) -> (junction 90968) [order 2]
            (junction 90966) -> (junction 90969) [order 2]
            (junction 90967) -> (junction 90970)
            (junction 90969) -> (junction 90968)
            (junction 90970) -> (junction 90969)
            (junction 90968) -> (junction 90971)
            (junction 90971) -> OpCl_doors.OpCl_3.Opening3.Button_detection1.BUTTON_DOWN.Button_DOWN_3 [order 1] : [PD3]
            OpCl_doors.OpCl_3.Opening3.Button_detection1.BUTTON_DOWN.Button_DOWN_3 -> (junction 90972)
            (junction 90972) -> OpCl_doors.OpCl_3.Opening3.Button_detection1.BUTTON_DOWN.First_but_3 [order 1] : [FIRST_BUT && not(RPC3)]
            OpCl_doors.OpCl_3.Opening3.Button_detection1.BUTTON_DOWN.First_but_3 -> (junction 90973)
            (junction 90971) -> (junction 90974) [order 2]
            (junction 90972) -> (junction 90975) [order 2]
            (junction 90973) -> (junction 90976)
            (junction 90975) -> (junction 90974)
            (junction 90976) -> (junction 90975)
          state BUTTON_CAR
            state Button_CAR_0
              en:
              BUTTON_CAR(1)=true;
              BUT_TEMP=0;
              LPC0=true;
              PUSHED=true;
              UPDATE=false;
              IN_LL=false; ET_LL=0;
            state First_but_0
              en:
              BUT_1=BUT_TEMP;
              FIRST_BUT=false;
            state Button_CAR_1
              en:
              BUTTON_CAR(2)=true;
              BUT_TEMP=1;
              LPC1=true;
              PUSHED=true;
              UPDATE=false;
              IN_LL=false; ET_LL=0;
            state First_but_1
              en:
              BUT_1=BUT_TEMP;
              FIRST_BUT=false;
            state Button_CAR_2
              en:
              BUTTON_CAR(3)=true;
              BUT_TEMP=2;
              LPC2=true;
              PUSHED=true;
              UPDATE=false;
              IN_LL=false; ET_LL=0;
            state First_but_2
              en:
              BUT_1=BUT_TEMP;
              FIRST_BUT=false;
            state Button_CAR_3
              en:
              BUTTON_CAR(4)=true;
              BUT_TEMP=3;
              LPC3=true;
              PUSHED=true;
              UPDATE=false;
              IN_LL=false; ET_LL=0;
            state First_but_3
              en:
              BUT_1=BUT_TEMP;
              FIRST_BUT=false;
            (default) -> (junction 91014)
            (junction 91014) -> OpCl_doors.OpCl_3.Opening3.Button_detection1.BUTTON_CAR.Button_CAR_0 [order 1] : [P0]
            OpCl_doors.OpCl_3.Opening3.Button_detection1.BUTTON_CAR.Button_CAR_0 -> (junction 91015)
            (junction 91015) -> OpCl_doors.OpCl_3.Opening3.Button_detection1.BUTTON_CAR.First_but_0 [order 1] : [FIRST_BUT && not(RPC0)]
            OpCl_doors.OpCl_3.Opening3.Button_detection1.BUTTON_CAR.First_but_0 -> (junction 91016)
            (junction 91014) -> (junction 91017) [order 2]
            (junction 91015) -> (junction 91018) [order 2]
            (junction 91016) -> (junction 91019)
            (junction 91018) -> (junction 91017)
            (junction 91019) -> (junction 91018)
            (junction 91017) -> (junction 91022)
            OpCl_doors.OpCl_3.Opening3.Button_detection1.BUTTON_CAR.Button_CAR_1 -> (junction 91020)
            (junction 91020) -> OpCl_doors.OpCl_3.Opening3.Button_detection1.BUTTON_CAR.First_but_1 [order 1] : [FIRST_BUT && not(RPC1)]
            OpCl_doors.OpCl_3.Opening3.Button_detection1.BUTTON_CAR.First_but_1 -> (junction 91021)
            (junction 91020) -> (junction 91024) [order 2]
            (junction 91021) -> (junction 91025)
            (junction 91022) -> OpCl_doors.OpCl_3.Opening3.Button_detection1.BUTTON_CAR.Button_CAR_1 [order 1] : [P1]
            (junction 91022) -> (junction 91023) [order 2]
            (junction 91024) -> (junction 91023)
            (junction 91025) -> (junction 91024)
            (junction 91023) -> (junction 91026)
            (junction 91026) -> OpCl_doors.OpCl_3.Opening3.Button_detection1.BUTTON_CAR.Button_CAR_2 [order 1] : [P2]
            OpCl_doors.OpCl_3.Opening3.Button_detection1.BUTTON_CAR.Button_CAR_2 -> (junction 91027)
            (junction 91027) -> OpCl_doors.OpCl_3.Opening3.Button_detection1.BUTTON_CAR.First_but_2 [order 1] : [FIRST_BUT && not(RPC2)]
            OpCl_doors.OpCl_3.Opening3.Button_detection1.BUTTON_CAR.First_but_2 -> (junction 91028)
            (junction 91026) -> (junction 91029) [order 2]
            (junction 91027) -> (junction 91030) [order 2]
            (junction 91028) -> (junction 91031)
            (junction 91030) -> (junction 91029)
            (junction 91031) -> (junction 91030)
            (junction 91029) -> (junction 91032)
            (junction 91032) -> OpCl_doors.OpCl_3.Opening3.Button_detection1.BUTTON_CAR.Button_CAR_3 [order 1] : [P3]
            OpCl_doors.OpCl_3.Opening3.Button_detection1.BUTTON_CAR.Button_CAR_3 -> (junction 91033)
            (junction 91033) -> OpCl_doors.OpCl_3.Opening3.Button_detection1.BUTTON_CAR.First_but_3 [order 1] : [FIRST_BUT && not(RPC3)]
            OpCl_doors.OpCl_3.Opening3.Button_detection1.BUTTON_CAR.First_but_3 -> (junction 91034)
            (junction 91032) -> (junction 91035) [order 2]
            (junction 91033) -> (junction 91036) [order 2]
            (junction 91034) -> (junction 91037)
            (junction 91036) -> (junction 91035)
            (junction 91037) -> (junction 91036)
          state BUTTON_UP
            state Button_UP_0
              en:
              BUTTON_UP(1)=true;
              BUT_TEMP=0;
              LPS0=true;
              PUSHED=true;
              UPDATE=false;
              IN_LL=false; ET_LL=0;
            state First_but_0
              en:
              BUT_1=BUT_TEMP;
              FIRST_BUT=false;
            state Button_UP_1
              en:
              BUTTON_UP(2)=true;
              BUT_TEMP=1;
              LPS1=true;
              PUSHED=true;
              UPDATE=false;
              IN_LL=false; ET_LL=0;
            state First_but_1
              en:
              BUT_1=BUT_TEMP;
              FIRST_BUT=false;
            state Button_UP_2
              en:
              BUTTON_UP(3)=true;
              BUT_TEMP=2;
              LPS2=true;
              PUSHED=true;
              UPDATE=false;
              IN_LL=false; ET_LL=0;
            state First_but_2
              en:
              BUT_1=BUT_TEMP;
              FIRST_BUT=false;
            (junction 91087) -> OpCl_doors.OpCl_3.Opening3.Button_detection1.BUTTON_UP.Button_UP_0 [order 1] : [PS0]
            OpCl_doors.OpCl_3.Opening3.Button_detection1.BUTTON_UP.Button_UP_0 -> (junction 91088)
            (junction 91088) -> OpCl_doors.OpCl_3.Opening3.Button_detection1.BUTTON_UP.First_but_0 [order 1] : [FIRST_BUT && not(RPC0)]
            OpCl_doors.OpCl_3.Opening3.Button_detection1.BUTTON_UP.First_but_0 -> (junction 91089)
            (default) -> (junction 91087)
            (junction 91087) -> (junction 91092) [order 2]
            (junction 91088) -> (junction 91090) [order 2]
            (junction 91089) -> (junction 91091)
            (junction 91091) -> (junction 91090)
            (junction 91090) -> (junction 91092)
            (junction 91092) -> (junction 91093)
            (junction 91093) -> OpCl_doors.OpCl_3.Opening3.Button_detection1.BUTTON_UP.Button_UP_1 [order 1] : [PS1]
            OpCl_doors.OpCl_3.Opening3.Button_detection1.BUTTON_UP.Button_UP_1 -> (junction 91094)
            (junction 91094) -> OpCl_doors.OpCl_3.Opening3.Button_detection1.BUTTON_UP.First_but_1 [order 1] : [FIRST_BUT && not(RPC1)]
            OpCl_doors.OpCl_3.Opening3.Button_detection1.BUTTON_UP.First_but_1 -> (junction 91095)
            (junction 91093) -> (junction 91096) [order 2]
            (junction 91094) -> (junction 91097) [order 2]
            (junction 91095) -> (junction 91098)
            (junction 91097) -> (junction 91096)
            (junction 91098) -> (junction 91097)
            (junction 91096) -> (junction 91100)
            OpCl_doors.OpCl_3.Opening3.Button_detection1.BUTTON_UP.First_but_2 -> (junction 91099)
            (junction 91099) -> (junction 91104)
            (junction 91100) -> OpCl_doors.OpCl_3.Opening3.Button_detection1.BUTTON_UP.Button_UP_2 [order 1] : [PS2]
            OpCl_doors.OpCl_3.Opening3.Button_detection1.BUTTON_UP.Button_UP_2 -> (junction 91101)
            (junction 91101) -> OpCl_doors.OpCl_3.Opening3.Button_detection1.BUTTON_UP.First_but_2 [order 1] : [FIRST_BUT && not(RPC2)]
            (junction 91100) -> (junction 91102) [order 2]
            (junction 91101) -> (junction 91103) [order 2]
            (junction 91103) -> (junction 91102)
            (junction 91104) -> (junction 91103)
          state Max_Min_assignment
            state Min_but
              en:
              BUTTON=MIN_BUT;
            state Max_but
              en:
              BUTTON=MAX_BUT;
            state First_but
              en:
              BUTTON=BUT_1;
            state Max_but1
              en:
              MAX_BUT=2;
            state Max_but2
              en:
              MAX_BUT=1;
            state Max_but3
              en:
              MAX_BUT=0;
            state Min_but1
              en:
              MIN_BUT=1;
            state Min_but2
              en:
              MIN_BUT=2;
            state Min_but3
              en:
              MIN_BUT=3;
            state MAX
              en:
              MAX_BUT=BUT_TEMP;
            state MIN
              en:
              MIN_BUT=BUT_TEMP;
            state Updating_button_0
              en:
              BUTTON=MAX_BUT;
            state Updating_button_1
              en:
              BUTTON=MIN_BUT;
            (junction 91142) -> OpCl_doors.OpCl_3.Opening3.Button_detection1.Max_Min_assignment.Min_but [order 1] : [(MAX_BUT-FLOOR)>(FLOOR-MIN_BUT)]
            OpCl_doors.OpCl_3.Opening3.Button_detection1.Max_Min_assignment.Min_but -> (junction 91143)
            (junction 91144) -> (junction 91142) [order 1] : [not(FLAG_STOP) && MOTION==2 && FLAG==3]
            (default) -> (junction 91144)
            (junction 91142) -> (junction 91145) [order 2]
            (junction 91143) -> (junction 91146)
            (junction 91144) -> (junction 91147) [order 2]
            (junction 91145) -> OpCl_doors.OpCl_3.Opening3.Button_detection1.Max_Min_assignment.Max_but [order 1] : [(MAX_BUT-FLOOR)<(FLOOR-MIN_BUT)]
            OpCl_doors.OpCl_3.Opening3.Button_detection1.Max_Min_assignment.Max_but -> (junction 91146)
            (junction 91145) -> OpCl_doors.OpCl_3.Opening3.Button_detection1.Max_Min_assignment.First_but [order 2]
            (junction 91146) -> (junction 91149)
            OpCl_doors.OpCl_3.Opening3.Button_detection1.Max_Min_assignment.First_but -> (junction 91148)
            (junction 91148) -> (junction 91147)
            (junction 91149) -> (junction 91148)
            (junction 91147) -> (junction 91150)
            (junction 91151) -> (junction 91152) [order 1] : [MOTION==0]
                | {MOTION=1;
                | UPDATE=true;}
            (junction 91152) -> OpCl_doors.OpCl_3.Opening3.Button_detection1.Max_Min_assignment.Max_but1 [order 1] : [BUTTON_UP(2)]
            OpCl_doors.OpCl_3.Opening3.Button_detection1.Max_Min_assignment.Max_but1 -> (junction 91153)
            (junction 91150) -> (junction 91151) [order 1] : [BUTTON==FLOOR && EXTEND]
                | {EXTEND=false;}
            (junction 91150) -> (junction 91164) [order 2]
            (junction 91151) -> (junction 91156) [order 2]
            (junction 91152) -> (junction 91154) [order 2]
            (junction 91153) -> (junction 91155)
            (junction 91154) -> OpCl_doors.OpCl_3.Opening3.Button_detection1.Max_Min_assignment.Max_but2 [order 1] : [BUTTON_UP(1)]
            OpCl_doors.OpCl_3.Opening3.Button_detection1.Max_Min_assignment.Max_but2 -> (junction 91155)
            (junction 91154) -> OpCl_doors.OpCl_3.Opening3.Button_detection1.Max_Min_assignment.Max_but3 [order 2]
            (junction 91155) -> (junction 91158)
            OpCl_doors.OpCl_3.Opening3.Button_detection1.Max_Min_assignment.Max_but3 -> (junction 91157)
            (junction 91157) -> (junction 91156)
            (junction 91158) -> (junction 91157)
            (junction 91156) -> (junction 91159)
            (junction 91159) -> (junction 91160) [order 1] : [MOTION==1]
                | {MOTION=0;
                | UPDATE=true;}
            (junction 91160) -> OpCl_doors.OpCl_3.Opening3.Button_detection1.Max_Min_assignment.Min_but1 [order 1] : [BUTTON_DOWN(1)]
            OpCl_doors.OpCl_3.Opening3.Button_detection1.Max_Min_assignment.Min_but1 -> (junction 91161)
            (junction 91159) -> (junction 91165) [order 2]
            (junction 91160) -> (junction 91162) [order 2]
            (junction 91161) -> (junction 91163)
            (junction 91162) -> OpCl_doors.OpCl_3.Opening3.Button_detection1.Max_Min_assignment.Min_but2 [order 1] : [BUTTON_DOWN(2)]
            OpCl_doors.OpCl_3.Opening3.Button_detection1.Max_Min_assignment.Min_but2 -> (junction 91163)
            (junction 91162) -> OpCl_doors.OpCl_3.Opening3.Button_detection1.Max_Min_assignment.Min_but3 [order 2]
            (junction 91163) -> (junction 91167)
            OpCl_doors.OpCl_3.Opening3.Button_detection1.Max_Min_assignment.Min_but3 -> (junction 91166)
            (junction 91165) -> (junction 91164)
            (junction 91166) -> (junction 91165)
            (junction 91167) -> (junction 91166)
            (junction 91164) -> (junction 91169)
            OpCl_doors.OpCl_3.Opening3.Button_detection1.Max_Min_assignment.MAX -> (junction 91168)
            (junction 91169) -> (junction 91170) [order 1] : [PUSHED]
            (junction 91170) -> (junction 91171) [order 1] : [not(BUT_TEMP==FLOOR) || not(MOTION==2)]
            (junction 91171) -> OpCl_doors.OpCl_3.Opening3.Button_detection1.Max_Min_assignment.MAX [order 1] : [MAX_BUT<BUT_TEMP && not(UPDATE)]
            (junction 91168) -> (junction 91173)
            (junction 91169) -> (junction 91183) [order 2]
            (junction 91170) -> (junction 91176) [order 2]
            (junction 91171) -> (junction 91172) [order 2]
            (junction 91173) -> (junction 91172)
            (junction 91172) -> (junction 91174)
            (junction 91174) -> OpCl_doors.OpCl_3.Opening3.Button_detection1.Max_Min_assignment.MIN [order 1] : [MIN_BUT>BUT_TEMP && not(UPDATE)]
            OpCl_doors.OpCl_3.Opening3.Button_detection1.Max_Min_assignment.MIN -> (junction 91175)
            (junction 91174) -> (junction 91177) [order 2]
            (junction 91175) -> (junction 91178)
            (junction 91177) -> (junction 91176)
            (junction 91178) -> (junction 91177)
            (junction 91176) -> (junction 91179)
            (junction 91179) -> OpCl_doors.OpCl_3.Opening3.Button_detection1.Max_Min_assignment.Updating_button_0 [order 1] : [MOTION==0]
            OpCl_doors.OpCl_3.Opening3.Button_detection1.Max_Min_assignment.Updating_button_0 -> (junction 91180)
            (junction 91179) -> (junction 91181) [order 2]
            (junction 91180) -> (junction 91182)
            (junction 91181) -> OpCl_doors.OpCl_3.Opening3.Button_detection1.Max_Min_assignment.Updating_button_1 [order 1] : [MOTION==1]
            OpCl_doors.OpCl_3.Opening3.Button_detection1.Max_Min_assignment.Updating_button_1 -> (junction 91182)
            (junction 91181) -> (junction 91184) [order 2]
            (junction 91182) -> (junction 91185)
            (junction 91184) -> (junction 91183)
            (junction 91185) -> (junction 91184)
          state GoTo_PositionControl
            en:
            BUTTON=BUT_TEMP;
            FLAG=2;
          state Emergency
            en:
            FLAG_EMG=true;
            FLAG=4;
          state Timer_EME
            state Set_tmr
              en:
              Q_EME=true;
            state Counting
              en:
              ET_EME= ET_EME + 1;
              Q_EME=false;
            state Set
              en:
              IN_EME=true;
              PT_EME=3;
            (junction 91275) -> OpCl_doors.OpCl_3.Opening3.Button_detection1.Timer_EME.Set_tmr [order 1] : [ET_EME==PT_EME]
            OpCl_doors.OpCl_3.Opening3.Button_detection1.Timer_EME.Set_tmr -> (junction 91276)
            OpCl_doors.OpCl_3.Opening3.Button_detection1.Timer_EME.Counting -> (junction 91275)
            (junction 91275) -> (junction 91276) [order 2]
            (default) -> OpCl_doors.OpCl_3.Opening3.Button_detection1.Timer_EME.Set
            OpCl_doors.OpCl_3.Opening3.Button_detection1.Timer_EME.Set -> (junction 91277)
            (junction 91277) -> OpCl_doors.OpCl_3.Opening3.Button_detection1.Timer_EME.Counting [order 1] : [ET_EME<PT_EME]
            (junction 91277) -> (junction 91276) [order 2]
          state Not_Emergency
            en:
            IN_EME=false;
            ET_EME=0;
          state SwitchingOFF_LEDs
            en:
            LPD3=false;
            LPD2=false;
            LPS2=false;
            LPD1=false;
            LPS1=false;
            LPS0=false;
          (default) -> (junction 90876)
          (junction 90876) -> (junction 90877) [order 1] : [FLAG==1 && not(PUSHED)]
              | {BUTTON=FLOOR;
              | BUT_TEMP=BUTTON;
              | BUT_1=FLOOR;}
          (junction 90877) -> OpCl_doors.OpCl_3.Opening3.Button_detection1.Timer_LL [order 1] : [not(FLAG_STOP)]
          OpCl_doors.OpCl_3.Opening3.Button_detection1.Save_energy -> (junction 90878)
          OpCl_doors.OpCl_3.Opening3.Button_detection1.Timer_LL -> OpCl_doors.OpCl_3.Opening3.Button_detection1.Save_energy
          (junction 90877) -> (junction 90880) [order 2]
          (junction 90876) -> (junction 90879) [order 2]
          (junction 90878) -> (junction 90881)
          (junction 90880) -> (junction 90879)
          (junction 90881) -> (junction 90880)
          (junction 90879) -> OpCl_doors.OpCl_3.Opening3.Button_detection1.BUTTON_CAR
          OpCl_doors.OpCl_3.Opening3.Button_detection1.BUTTON_UP -> OpCl_doors.OpCl_3.Opening3.Button_detection1.BUTTON_DOWN
          OpCl_doors.OpCl_3.Opening3.Button_detection1.BUTTON_DOWN -> OpCl_doors.OpCl_3.Opening3.Button_detection1.Max_Min_assignment
          OpCl_doors.OpCl_3.Opening3.Button_detection1.Max_Min_assignment -> (junction 90882)
          OpCl_doors.OpCl_3.Opening3.Button_detection1.BUTTON_CAR -> OpCl_doors.OpCl_3.Opening3.Button_detection1.BUTTON_UP
          (junction 90882) -> (junction 90884)
          (junction 90884) -> (junction 90883)
          (junction 90883) -> (junction 90886)
          OpCl_doors.OpCl_3.Opening3.Button_detection1.GoTo_PositionControl -> (junction 90885)
          (junction 90886) -> (junction 90887) [order 1] : [FLAG==1]
          (junction 90887) -> OpCl_doors.OpCl_3.Opening3.Button_detection1.GoTo_PositionControl [order 1] : [PUSHED]
          (junction 90885) -> (junction 90889)
          (junction 90886) -> (junction 90897) [order 2]
          (junction 90887) -> (junction 90888) [order 2]
          (junction 90889) -> (junction 90888)
          (junction 90888) -> (junction 90891)
          OpCl_doors.OpCl_3.Opening3.Button_detection1.Emergency -> (junction 90890)
          (junction 90891) -> OpCl_doors.OpCl_3.Opening3.Button_detection1.Timer_EME [order 1] : [STOP]
              | {IN_LL=false; ET_LL=0;FLAG=1;}
          OpCl_doors.OpCl_3.Opening3.Button_detection1.Timer_EME -> (junction 90892)
          (junction 90892) -> OpCl_doors.OpCl_3.Opening3.Button_detection1.Emergency [order 1] : [Q_EME]
          (junction 90890) -> (junction 90894)
          (junction 90891) -> OpCl_doors.OpCl_3.Opening3.Button_detection1.Not_Emergency [order 2]
          (junction 90892) -> (junction 90893) [order 2]
          (junction 90894) -> (junction 90893)
          (junction 90893) -> (junction 90896)
          OpCl_doors.OpCl_3.Opening3.Button_detection1.Not_Emergency -> (junction 90896)
          OpCl_doors.OpCl_3.Opening3.Button_detection1.SwitchingOFF_LEDs -> (junction 90895)
          (junction 90896) -> OpCl_doors.OpCl_3.Opening3.Button_detection1.SwitchingOFF_LEDs [order 1] : [FLAG_STOP && FLAG==2]
          (junction 90895) -> (junction 90899)
          (junction 90896) -> (junction 90898) [order 2]
          (junction 90898) -> (junction 90897)
          (junction 90899) -> (junction 90898)
        state Opening1
          en:AP3=true;
        state Reset
          state Reset_0
            en:
            LPS0=false;
            BUTTON_CAR(1)=false;
            BUTTON_UP(1)=false;
          state Reset_1
            en:
            LPS1=false;
            LPD1=false;
            BUTTON_CAR(2)=false;
            BUTTON_UP(2)=false;
            BUTTON_DOWN(2)=false;
          state Reset_2
            en:
            LPS2=false;
            LPD2=false;
            BUTTON_CAR(3)=false;
            BUTTON_UP(3)=false;
            BUTTON_DOWN(3)=false;
          state Reset_3
            en:
            LPD3=false;
            BUTTON_CAR(4)=false;
            BUTTON_DOWN(4)=false;
          (default) -> (junction 91293)
          (junction 91293) -> OpCl_doors.OpCl_3.Opening3.Reset.Reset_0 [order 1] : [FLOOR==0]
          OpCl_doors.OpCl_3.Opening3.Reset.Reset_0 -> (junction 91294)
          (junction 91293) -> (junction 91295) [order 2]
          (junction 91294) -> (junction 91296)
          (junction 91295) -> OpCl_doors.OpCl_3.Opening3.Reset.Reset_1 [order 1] : [FLOOR==1]
          OpCl_doors.OpCl_3.Opening3.Reset.Reset_1 -> (junction 91296)
          (junction 91295) -> (junction 91297) [order 2]
          (junction 91296) -> (junction 91298)
          (junction 91297) -> OpCl_doors.OpCl_3.Opening3.Reset.Reset_2 [order 1] : [FLOOR==2]
          OpCl_doors.OpCl_3.Opening3.Reset.Reset_2 -> (junction 91298)
          (junction 91297) -> (junction 91299) [order 2]
          (junction 91298) -> (junction 91300)
          (junction 91299) -> OpCl_doors.OpCl_3.Opening3.Reset.Reset_3 [order 1] : [FLOOR==3]
          OpCl_doors.OpCl_3.Opening3.Reset.Reset_3 -> (junction 91300)
          (junction 91299) -> (junction 91301) [order 2]
          (junction 91300) -> (junction 91302)
          (junction 91302) -> (junction 91301)
        state Stop_Opening1
          en: AP3=false;
          FLAG_OD=true;
          IN_cl=false;
          ET_cl=0;
        (junction 90290) -> (junction 90291)
        (junction 90291) -> (junction 90292) [order 1] : [not(OBS) ]
        (junction 90294) -> OpCl_doors.OpCl_3.Opening3.Opening [order 1] : [not(PA3)]
        (junction 90292) -> (junction 90293) [order 2]
        (junction 90293) -> OpCl_doors.OpCl_3.Opening3.Timer_open
        OpCl_doors.OpCl_3.Opening3.Timer_open -> (junction 90294)
        (default) -> OpCl_doors.OpCl_3.Opening3.People_IN
        (junction 90291) -> (junction 90295) [order 2]
        (junction 90292) -> OpCl_doors.OpCl_3.Opening3.Button_detection [order 1] : [not(FLAG==4)]
        (junction 90297) -> (junction 90293)
        (junction 90299) -> (junction 90290)
        (junction 90294) -> OpCl_doors.OpCl_3.Opening3.Stop_Opening [order 2]
        OpCl_doors.OpCl_3.Opening3.People_IN -> OpCl_doors.OpCl_3.Opening3.People_OUT
        OpCl_doors.OpCl_3.Opening3.Opening -> (junction 90304)
        (junction 90295) -> (junction 90296) [order 2]
        (junction 90295) -> OpCl_doors.OpCl_3.Opening3.Button_detection1 [order 1] : [not(FLAG==4)]
        (junction 90296) -> (junction 90301)
        OpCl_doors.OpCl_3.Opening3.Button_detection -> (junction 90297)
        OpCl_doors.OpCl_3.Opening3.People_OUT -> (junction 90298)
        OpCl_doors.OpCl_3.Opening3.Button_detection1 -> (junction 90300)
        (junction 90301) -> (junction 90300)
        (junction 90298) -> (junction 90299) [order 2]
        (junction 90298) -> OpCl_doors.OpCl_3.Opening3.Reset [order 1] : [not(FLAG==4)]
        (junction 90300) -> (junction 90302)
        (junction 90308) -> (junction 90299)
        OpCl_doors.OpCl_3.Opening3.Stop_Opening -> (junction 90303)
        (junction 90302) -> OpCl_doors.OpCl_3.Opening3.Opening1 [order 1] : [not(PA3)]
        (junction 90302) -> OpCl_doors.OpCl_3.Opening3.Stop_Opening1 [order 2]
        (junction 90304) -> (junction 90303)
        (junction 90303) -> (junction 90306)
        OpCl_doors.OpCl_3.Opening3.Opening1 -> (junction 90305)
        OpCl_doors.OpCl_3.Opening3.Reset -> (junction 90307)
        OpCl_doors.OpCl_3.Opening3.Stop_Opening1 -> (junction 90305)
        (junction 90305) -> (junction 90306)
        (junction 90307) -> (junction 90308)
      (default) -> (junction 13058)
      (junction 13058) -> (junction 13057) [order 1] : [FLAG_OD]
      (junction 13057) -> OpCl_doors.OpCl_3.Closing3 [order 1] : [not(SWITCH) && not(STOP) && WEIGHT<=320 && not(PD3 || P3)]
      OpCl_doors.OpCl_3.Closing3 -> (junction 30497)
      (junction 13058) -> OpCl_doors.OpCl_3.Opening3 [order 2]
      (junction 13057) -> OpCl_doors.OpCl_3.StopClosing [order 2]
      (junction 30497) -> (junction 30500)
      OpCl_doors.OpCl_3.StopClosing -> (junction 30498)
      (junction 30500) -> (junction 30498)
      (junction 30498) -> (junction 30499)
      OpCl_doors.OpCl_3.Opening3 -> (junction 30499)
    OpCl_doors.Button_detection -> (junction 12501)
    (junction 12501) -> OpCl_0 [order 1] : [FLOOR==0]
    OpCl_0 -> (junction 30451)
    (default) -> OpCl_doors.Button_detection
    (junction 12501) -> (junction 30445) [order 2]
    (junction 30451) -> (junction 30453)
    (junction 30445) -> OpCl_1 [order 1] : [FLOOR==1]
    OpCl_1 -> (junction 30453)
    (junction 30445) -> (junction 30447) [order 2]
    (junction 30453) -> (junction 30456)
    (junction 30447) -> OpCl_2 [order 1] : [FLOOR==2]
    OpCl_2 -> (junction 30456)
    (junction 30447) -> (junction 30449) [order 2]
    (junction 30456) -> (junction 30461)
    (junction 30449) -> OpCl_3 [order 1] : [FLOOR==3]
    OpCl_3 -> (junction 30461)
    (junction 30449) -> (junction 30459) [order 2]
    (junction 30461) -> (junction 30460)
    (junction 30460) -> (junction 30459)
  state Emergency
    state BLK_Eme
      %BLK(LPS0)
      %BLK(LPD1)
      %BLK(LPS1)
      %BLK(LPD2)
      %BLK(LPS2)
      %BLK(LPD3)
    state REC
      %BLK(LL)
    state FIRST
      en:
      LPC0=false;
      LPC1=false;
      LPC2=false;
      LPC3=false;
      FIRST=false;
    state Replacing
      en:
      SCENDI=true;
    state Replaced
      en:
      SCENDI=false;
    state Doors
      state FLOOR_0
        en: CP0=false;
      state Opening0
        state Opening
          en:AP0=Q_op;
        state People_IN
          state Check_People_IN
            en:
            COUNTER_IN=false;
          state People_KID_IN
            en:
            WEIGHT=WEIGHT+30;
            KIDS=KIDS+1;
          state People_WOMAN_IN
            en:
            WEIGHT=WEIGHT+55;
            WOMEN=WOMEN+1;
          state People_MAN_IN
            en:
            WEIGHT=WEIGHT+75;
            MEN=MEN+1;
          state People_FATGUY_IN
            en:
            WEIGHT=WEIGHT+100;
            FATGUYS=FATGUYS+1;
          state Re_Ready_IN
            en:
            COUNTER_IN=true;
          (default) -> (junction 91383)
          (junction 91383) -> Emergency.Doors.Opening0.People_IN.Check_People_IN [order 1] : [COUNTER_IN]
          Emergency.Doors.Opening0.People_IN.Check_People_IN -> (junction 91384)
          (junction 91384) -> Emergency.Doors.Opening0.People_IN.People_KID_IN [order 1] : [KID_IN]
          Emergency.Doors.Opening0.People_IN.People_KID_IN -> (junction 91385)
          (junction 91383) -> (junction 91392) [order 2]
          (junction 91384) -> (junction 91386) [order 2]
          (junction 91385) -> (junction 91387)
          (junction 91386) -> Emergency.Doors.Opening0.People_IN.People_WOMAN_IN [order 1] : [WOMAN_IN]
          Emergency.Doors.Opening0.People_IN.People_WOMAN_IN -> (junction 91387)
          (junction 91386) -> (junction 91388) [order 2]
          (junction 91387) -> (junction 91389)
          (junction 91388) -> Emergency.Doors.Opening0.People_IN.People_MAN_IN [order 1] : [MAN_IN]
          Emergency.Doors.Opening0.People_IN.People_MAN_IN -> (junction 91389)
          (junction 91388) -> (junction 91390) [order 2]
          (junction 91389) -> (junction 91391)
          (junction 91390) -> Emergency.Doors.Opening0.People_IN.People_FATGUY_IN [order 1] : [FATGUY_IN]
          Emergency.Doors.Opening0.People_IN.People_FATGUY_IN -> (junction 91391)
          (junction 91390) -> (junction 91393) [order 2]
          (junction 91391) -> (junction 91394)
          (junction 91393) -> (junction 91392)
          (junction 91394) -> (junction 91393)
          (junction 91392) -> (junction 91395)
          (junction 91395) -> Emergency.Doors.Opening0.People_IN.Re_Ready_IN [order 1] : [not(KID_IN|| WOMAN_IN || MAN_IN || FATGUY_IN)]
          (junction 91395) -> (junction 91396) [order 2]
          Emergency.Doors.Opening0.People_IN.Re_Ready_IN -> (junction 91397)
          (junction 91397) -> (junction 91396)
        state Timer_open
          state Set_tmr
            en: Q_op=true;
          state Set
            en:PT_op=2;
            IN_op=true;
          state Counting
            en:ET_op = ET_op + 1;
            Q_op=false;
          (junction 91432) -> Emergency.Doors.Opening0.Timer_open.Set_tmr [order 1] : [ET_op==PT_op]
          Emergency.Doors.Opening0.Timer_open.Set_tmr -> (junction 91433)
          (default) -> Emergency.Doors.Opening0.Timer_open.Set
          Emergency.Doors.Opening0.Timer_open.Counting -> (junction 91432)
          (junction 91432) -> (junction 91433) [order 2]
          Emergency.Doors.Opening0.Timer_open.Set -> (junction 91434)
          (junction 91434) -> Emergency.Doors.Opening0.Timer_open.Counting [order 1] : [ET_op<PT_op]
          (junction 91434) -> (junction 91433) [order 2]
        state Stop_Opening
          en:AP0=false;
          FLAG_OD=true;
          OBS=true;
          IN_op=false;
          ET_op=0;
        state People_OUT
          state Check_People_OUT
            en:
            COUNTER_OUT=false;
          state People_KID_OUT
            en:
            WEIGHT=WEIGHT-30;
            KIDS=KIDS-1;
          state People_WOMAN_OUT
            en:
            WEIGHT=WEIGHT-55;
            WOMEN=WOMEN-1;
          state People_MAN_OUT
            en:
            WEIGHT=WEIGHT-75;
            MEN=MEN-1;
          state People_FATGUY_OUT
            en:
            WEIGHT=WEIGHT-100;
            FATGUYS=FATGUYS-1;
          state Re_Ready_OUT
            en:
            COUNTER_OUT=true;
          (default) -> (junction 91448)
          (junction 91448) -> Emergency.Doors.Opening0.People_OUT.Check_People_OUT [order 1] : [COUNTER_OUT]
          Emergency.Doors.Opening0.People_OUT.Check_People_OUT -> (junction 91449)
          (junction 91449) -> Emergency.Doors.Opening0.People_OUT.People_KID_OUT [order 1] : [KID_OUT && KIDS>0 ]
          Emergency.Doors.Opening0.People_OUT.People_KID_OUT -> (junction 91450)
          (junction 91448) -> (junction 91457) [order 2]
          (junction 91449) -> (junction 91451) [order 2]
          (junction 91450) -> (junction 91452)
          (junction 91451) -> Emergency.Doors.Opening0.People_OUT.People_WOMAN_OUT [order 1] : [WOMAN_OUT && WOMEN>0]
          Emergency.Doors.Opening0.People_OUT.People_WOMAN_OUT -> (junction 91452)
          (junction 91452) -> (junction 91454)
          (junction 91451) -> (junction 91453) [order 2]
          (junction 91453) -> Emergency.Doors.Opening0.People_OUT.People_MAN_OUT [order 1] : [MAN_OUT && MEN>0]
          Emergency.Doors.Opening0.People_OUT.People_MAN_OUT -> (junction 91454)
          (junction 91453) -> (junction 91455) [order 2]
          (junction 91454) -> (junction 91456)
          (junction 91455) -> Emergency.Doors.Opening0.People_OUT.People_FATGUY_OUT [order 1] : [FATGUY_OUT && FATGUYS>0]
          Emergency.Doors.Opening0.People_OUT.People_FATGUY_OUT -> (junction 91456)
          (junction 91455) -> (junction 91458) [order 2]
          (junction 91456) -> (junction 91459)
          (junction 91458) -> (junction 91457)
          (junction 91459) -> (junction 91458)
          (junction 91457) -> (junction 91460)
          (junction 91460) -> Emergency.Doors.Opening0.People_OUT.Re_Ready_OUT [order 1] : [not(KID_OUT || WOMAN_OUT || MAN_OUT || FATGUY_OUT)]
          (junction 91460) -> (junction 91461) [order 2]
          Emergency.Doors.Opening0.People_OUT.Re_Ready_OUT -> (junction 91462)
          (junction 91462) -> (junction 91461)
        state Button_detection
          state Save_energy
            en:
            LL=not(Q_LL);
          state Timer_LL
            state Set_tmr
              en:
              Q_LL=true;
            state Counting
              en:
              ET_LL= ET_LL + 1;
              Q_LL=false;
            state Set
              en:
              IN_LL=true;
              PT_LL=10;
            (junction 91565) -> Emergency.Doors.Opening0.Button_detection.Timer_LL.Set_tmr [order 1] : [ET_LL==PT_LL]
            Emergency.Doors.Opening0.Button_detection.Timer_LL.Set_tmr -> (junction 91566)
            Emergency.Doors.Opening0.Button_detection.Timer_LL.Counting -> (junction 91565)
            (junction 91565) -> (junction 91566) [order 2]
            (default) -> Emergency.Doors.Opening0.Button_detection.Timer_LL.Set
            Emergency.Doors.Opening0.Button_detection.Timer_LL.Set -> (junction 91567)
            (junction 91567) -> Emergency.Doors.Opening0.Button_detection.Timer_LL.Counting [order 1] : [ET_LL<PT_LL]
            (junction 91567) -> (junction 91566) [order 2]
          state BUTTON_DOWN
            state Button_DOWN_1
              en:
              BUTTON_DOWN(2)=true;
              BUT_TEMP=1;
              LPD1=true;
              PUSHED=true;
              UPDATE=false;
              IN_LL=false; ET_LL=0;
            state First_but_1
              en:
              BUT_1=BUT_TEMP;
              FIRST_BUT=false;
            state Button_DOWN_2
              en:
              BUTTON_DOWN(3)=true;
              BUT_TEMP=2;
              LPD2=true;
              PUSHED=true;
              UPDATE=false;
              IN_LL=false; ET_LL=0;
            state First_but_2
              en:
              BUT_1=BUT_TEMP;
              FIRST_BUT=false;
            state Button_DOWN_3
              en:
              BUTTON_DOWN(4)=true;
              BUT_TEMP=3;
              LPD3=true;
              PUSHED=true;
              UPDATE=false;
              IN_LL=false; ET_LL=0;
            state First_but_3
              en:
              BUT_1=BUT_TEMP;
              FIRST_BUT=false;
            (default) -> (junction 91580)
            (junction 91580) -> Emergency.Doors.Opening0.Button_detection.BUTTON_DOWN.Button_DOWN_1 [order 1] : [PD1]
            Emergency.Doors.Opening0.Button_detection.BUTTON_DOWN.Button_DOWN_1 -> (junction 91581)
            (junction 91581) -> Emergency.Doors.Opening0.Button_detection.BUTTON_DOWN.First_but_1 [order 1] : [FIRST_BUT && not(RPC1)]
            Emergency.Doors.Opening0.Button_detection.BUTTON_DOWN.First_but_1 -> (junction 91582)
            (junction 91580) -> (junction 91583) [order 2]
            (junction 91581) -> (junction 91584) [order 2]
            (junction 91582) -> (junction 91585)
            (junction 91584) -> (junction 91583)
            (junction 91585) -> (junction 91584)
            (junction 91583) -> (junction 91586)
            (junction 91586) -> Emergency.Doors.Opening0.Button_detection.BUTTON_DOWN.Button_DOWN_2 [order 1] : [PD2]
            Emergency.Doors.Opening0.Button_detection.BUTTON_DOWN.Button_DOWN_2 -> (junction 91587)
            (junction 91587) -> Emergency.Doors.Opening0.Button_detection.BUTTON_DOWN.First_but_2 [order 1] : [FIRST_BUT && not(RPC2)]
            Emergency.Doors.Opening0.Button_detection.BUTTON_DOWN.First_but_2 -> (junction 91588)
            (junction 91586) -> (junction 91589) [order 2]
            (junction 91587) -> (junction 91590) [order 2]
            (junction 91588) -> (junction 91591)
            (junction 91590) -> (junction 91589)
            (junction 91591) -> (junction 91590)
            (junction 91589) -> (junction 91592)
            (junction 91592) -> Emergency.Doors.Opening0.Button_detection.BUTTON_DOWN.Button_DOWN_3 [order 1] : [PD3]
            Emergency.Doors.Opening0.Button_detection.BUTTON_DOWN.Button_DOWN_3 -> (junction 91593)
            (junction 91593) -> Emergency.Doors.Opening0.Button_detection.BUTTON_DOWN.First_but_3 [order 1] : [FIRST_BUT && not(RPC3)]
            Emergency.Doors.Opening0.Button_detection.BUTTON_DOWN.First_but_3 -> (junction 91594)
            (junction 91592) -> (junction 91595) [order 2]
            (junction 91593) -> (junction 91596) [order 2]
            (junction 91594) -> (junction 91597)
            (junction 91596) -> (junction 91595)
            (junction 91597) -> (junction 91596)
          state BUTTON_CAR
            state Button_CAR_0
              en:
              BUTTON_CAR(1)=true;
              BUT_TEMP=0;
              LPC0=true;
              PUSHED=true;
              UPDATE=false;
              IN_LL=false; ET_LL=0;
            state First_but_0
              en:
              BUT_1=BUT_TEMP;
              FIRST_BUT=false;
            state Button_CAR_1
              en:
              BUTTON_CAR(2)=true;
              BUT_TEMP=1;
              LPC1=true;
              PUSHED=true;
              UPDATE=false;
              IN_LL=false; ET_LL=0;
            state First_but_1
              en:
